simulink model "controller_dev_sg_RCP"  (R2018b)
settings: configuration reference "Active" (kept outside this file)
model workspace (MAT data in the model file):
  m = 1000
undefined symbols (not defined in the file or in its folder): C, tS, TUMHealthStatus, TUMVehicleState
libraries: xpcrtudplib x6, simulink x6, canmsglib x6, etargetslib x5, misc x4, speedgoatlib_IO614 x3, slrtlib x2
(part 2 of 3)

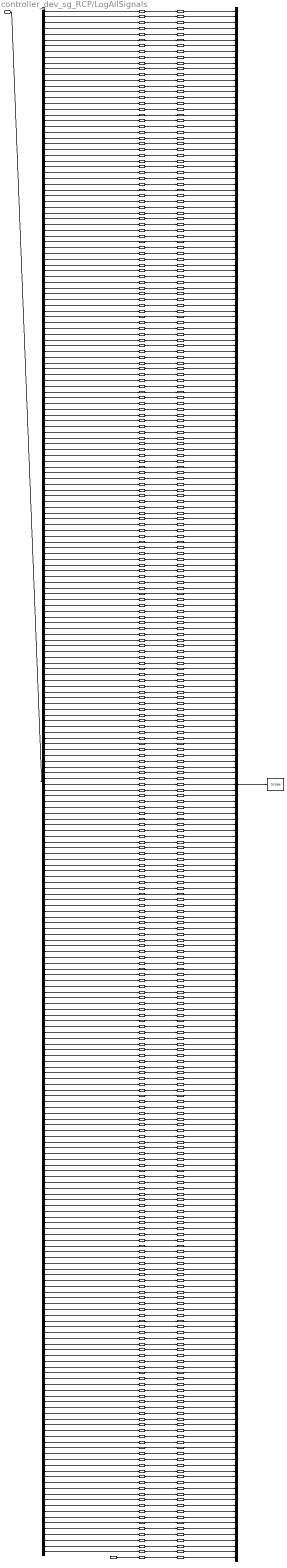
== system controller_dev_sg_RCP/LogAllSignals ==
  debugIn : Inport  OutDataTypeStr=Bus: mvdc_vehicle_dynamics_control_debug
  BusOutput : BusSelector  OutputSignals=ErrorCode,mvdc_path_feedback_debug.BarriersL_x_m,mvdc_path_feedback_debug.BarriersL_y_m,mvdc_path_feedback_debug.BarriersR_x_m,mvdc_path_feedback_debug.BarriersR_y_m,mvdc_path_feedback_debug.LeftDistance_m,mvdc_path_feedback_debug.RightDistance_m,mvdc_path_feedback_debug.Lat_FB_Barriers,mvdc_path_feedback_debug.Lat_FB_Sum_KappaReq_radpm,mvdc_path_feedback_debug.Lat_FB_Position,mvdc_path_feedback_debug.Lat_FB_Heading,mvdc_path_feedback_debug.Lat_LatPosError_m,mvdc_path_feedback_debug.Lat_LatPosError_DerAna_mps,mvdc_path_feedback_debug.Lat_LatPosError_DerNum_mps,mvdc_path_feedback_debug.Lat_FF_Kappa_KappaReq_radpm,mvdc_path_feedback_debug.Lat_FF_FIR_radpm,mvdc_path_feedback_debug.Lat_all_KappaReq_radpm,mvdc_path_matching_debug.PerformanceTrajOK_b,mvdc_path_matching_debug.EmergencyTrajOK_b,mvdc_path_matching_debug.PathPos.s_m,mvdc_path_matching_debug.PathPos.d_m,mvdc_path_matching_debug.PathPos.psi_rad,mvdc_path_matching_debug.ActualPathPoint.LapCnt,mvdc_path_matching_debug.ActualPathPoint.TrajCnt,mvdc_path_matching_debug.ActualPathPoint.s_m,mvdc_path_matching_debug.ActualPathPoint.x_m,mvdc_path_matching_debug.ActualPathPoint.y_m,mvdc_path_matching_debug.ActualPathPoint.psi_rad,mvdc_path_matching_debug.ActualPathPoint.kappa_radpm,mvdc_path_matching_debug.ActualPathPoint.kappaFF_radpm,mvdc_path_matching_debug.ActualPathPoint.v_mps,mvdc_path_matching_debug.ActualPathPoint.ax_mps2,mvdc_path_matching_debug.ActualPathPoint.axFF_mps2,mvdc_path_matching_debug.ActualPathPoint.Delta_rad,mvdc_path_matching_debug.ActualPathPoint.DriveForce_N,mvdc_trajectory_driver_debug.ParkBrakeActive,mvdc_trajectory_driver_debug.DriverStatus,mvdc_trajectory_driver_debug.EnablePathMatching,mvdc_trajectory_driver_debug.EnableDriving,mvdc_trajectory_driver_debug.PathMatchingStatus,mvdc_trajectory_driver_debug.Strategy_Status,mvdc_trajectory_driver_debug.Trajectories_CommsStatus,mvdc_trajectory_driver_debug.Strategy_CommsStatus,mvdc_trajectory_driver_perf.LapTime_s,mvdc_trajectory_driver_perf.e_lateral_m,mvdc_trajectory_driver_perf.eRMS_lateral_m,mvdc_trajectory_driver_perf.ePeak_lateral_m,mvdc_trajectory_driver_perf.e_heading_rad,mvdc_trajectory_driver_perf.eRMS_heading_rad,mvdc_trajectory_driver_perf.ePeak_heading_rad,mvdc_trajectory_driver_perf.e_v_mps,mvdc_trajectory_driver_perf.eRMS_v_mps,mvdc_trajectory_driver_perf.ePeak_v_mps,mvdc_trajectory_driver_perf.e_kappa_radpm,mvdc_trajectory_driver_perf.eRMS_kappa_radpm,mvdc_trajectory_driver_perf.ePeak_kappa_radpm,mvdc_curvvel_tracking_debug.Curv_TargetAy_mps2,mvdc_curvvel_tracking_debug.Curv_all_KappaReq_radpm,mvdc_curvvel_tracking_debug.Curv_FB_Dist_DeltaReq_rad,mvdc_curvvel_tracking_debug.Curv_FB_Diff_DeltaReq_rad,mvdc_curvvel_tracking_debug.Curv_FF_Kappa_DeltaReq_rad,mvdc_curvvel_tracking_debug.Curv_USComp_DeltaReq_rad,mvdc_curvvel_tracking_debug.Curv_CurvError_radpm,mvdc_curvvel_tracking_debug.Curv_TargetCurv_radpm,mvdc_curvvel_tracking_debug.Long_FB_Dist_FxReq_N,mvdc_curvvel_tracking_debug.Long_FF_Dist_FxReq_N,mvdc_curvvel_tracking_debug.Long_FB_VelDiff_FxReq_N,mvdc_curvvel_tracking_debug.Long_FF_Traj_FxReq_N,mvdc_curvvel_tracking_debug.Long_VelError_mps,mvdc_curvvel_tracking_debug.Long_TargetSpeed_mps,mvdc_curvvel_tracking_debug.Long_axTarget_mps2,mvdc_curvvel_tracking_debug.Req_Delta_rad,mvdc_curvvel_tracking_debug.Req_Fx_N,mvdc_curvvel_tracking_debug.ControlState,mvdc_curvvel_tracking_debug.EnableDriving,mvdc_curvvel_tracking_debug.EnableEmergency,mvdc_curvvel_tracking_debug.TCCorrectiveForce_N,mvdc_curvvel_tracking_debug.TCSlipDifference_perc,mvdc_curvvel_tracking_debug.TCProportionalForce_N,mvdc_curvvel_tracking_debug.TCIntegralForce_N,mvdc_curvvel_tracking_debug.MaximumLongForce_N,mvdc_exactlin_feedback_debug.VelocityError_mps,mvdc_exactlin_feedback_debug.LongAccTarget_mps2,mvdc_exactlin_feedback_debug.LatError_m,mvdc_exactlin_feedback_debug.LatErrorDer_mps,mvdc_exactlin_feedback_debug.LatAccTarget_mps2,mvdc_exactlin_feedback_debug.EstimateAlphaF_rad,mvdc_exactlin_feedback_debug.EstimateAlphaR_rad,mvdc_exactlin_feedback_debug.EstimateFyF_N,mvdc_exactlin_feedback_debug.EstimateFyR_N,mvdc_exactlin_feedback_debug.RequestDelta_rad,mvdc_exactlin_feedback_debug.RequestFx_N,mvdc_state_estimation_debug.StateEstimate.SE_Status,mvdc_state_estimation_debug.StateEstimate.SE_State,mvdc_state_estimation_debug.StateEstimate.Pos.x_m,mvdc_state_estimation_debug.StateEstimate.Pos.y_m,mvdc_state_estimation_debug.StateEstimate.Pos.psi_rad,mvdc_state_estimation_debug.StateEstimate.z_m,mvdc_state_estimation_debug.StateEstimate.PosAccuracy,mvdc_state_estimation_debug.StateEstimate.VelAccuracy,mvdc_state_estimation_debug.StateEstimate.dPsi_radps,mvdc_state_estimation_debug.StateEstimate.vx_mps,mvdc_state_estimation_debug.StateEstimate.vy_mps,mvdc_state_estimation_debug.StateEstimate.v_mps,mvdc_state_estimation_debug.StateEstimate.beta_rad,mvdc_state_estimation_debug.StateEstimate.ax_mps2,mvdc_state_estimation_debug.StateEstimate.ay_mps2,mvdc_state_estimation_debug.StateEstimate.psi_vel_rad,mvdc_state_estimation_debug.StateEstimate.kappa_radpm,mvdc_state_estimation_debug.StateEstimate.dBeta_radps,mvdc_state_estimation_debug.StateEstimate.ddPsi_radps2,mvdc_state_estimation_debug.StateEstimate.ax_vel_mps2,mvdc_state_estimation_debug.StateEstimate.ay_vel_mps2,mvdc_state_estimation_debug.StateEstimate.lambdaFL_perc,mvdc_state_estimation_debug.StateEstimate.lambdaFR_perc,mvdc_state_estimation_debug.StateEstimate.lambdaRL_perc,mvdc_state_estimation_debug.StateEstimate.lambdaRR_perc,mvdc_state_estimation_debug.StateEstimate.alphaFL_rad,mvdc_state_estimation_debug.StateEstimate.alphaFR_rad,mvdc_state_estimation_debug.StateEstimate.alphaRL_rad,mvdc_state_estimation_debug.StateEstimate.alphaRR_rad,mvdc_state_estimation_debug.StateEstimate.DiffFRAlpha_rad,mvdc_state_estimation_debug.Residuals.res_xLoc1_m,mvdc_state_estimation_debug.Residuals.res_yLoc1_m,mvdc_state_estimation_debug.Residuals.res_psiLoc1_rad,mvdc_state_estimation_debug.Residuals.res_xLoc2_m,mvdc_state_estimation_debug.Residuals.res_yLoc2_m,mvdc_state_estimation_debug.Residuals.res_psiLoc2_rad,mvdc_state_estimation_debug.Residuals.res_vxVel1_mps,mvdc_state_estimation_debug.Residuals.res_vyVel1_mps,mvdc_state_estimation_debug.Residuals.res_vxVel2_mps,mvdc_state_estimation_debug.Residuals.res_vyVel2_mps,mvdc_state_estimation_debug.Residuals.res_dPsi1_radps,mvdc_state_estimation_debug.Residuals.res_dPsi2_radps,mvdc_state_estimation_debug.Residuals.res_sLoc1_m,mvdc_state_estimation_debug.Residuals.res_dLoc1_m,mvdc_state_estimation_debug.Residuals.res_sLoc2_m,mvdc_state_estimation_debug.Residuals.res_dLoc2_m,mvdc_state_estimation_debug.Diagnosis.valid_Loc1_b,mvdc_state_estimation_debug.Diagnosis.valid_Loc2_b,mvdc_state_estimation_debug.Diagnosis.valid_Vel1_b,mvdc_state_estimation_debug.Diagnosis.valid_Vel2_b,mvdc_state_estimation_debug.Diagnosis.valid_IMU1_b,mvdc_state_estimation_debug.Diagnosis.valid_IMU2_b,mvdc_state_estimation_debug.Diagnosis.fail_Loc1_b,mvdc_state_estimation_debug.Diagnosis.fail_Loc2_b,mvdc_state_estimation_debug.Diagnosis.fail_Vel1_b,mvdc_state_estimation_debug.Diagnosis.fail_Vel2_b,mvdc_state_estimation_debug.Diagnosis.fail_IMU1_b,mvdc_state_estimation_debug.Diagnosis.fail_IMU2_b,mvdc_state_estimation_debug.Odom.Position.x_m,mvdc_state_estimation_debug.Odom.Position.y_m,mvdc_state_estimation_debug.Odom.Position.psi_rad,mvdc_state_estimation_debug.Odom.Valid_b,mloc_statemachine_debug.Hardware_Status,mloc_statemachine_debug.AIDriver_Status,mloc_statemachine_debug.ParkBrakeApplied_b,mloc_statemachine_debug.VehicleReady2Drive,mloc_statemachine_debug.StateEstimation_Status,mloc_statemachine_debug.VehicleSafeStandstill,mloc_statemachine_debug.Driver_Status,mloc_statemachine_debug.VehicleUnresponsive,mloc_statemachine_debug.TUMVehicleState,mloc_statemachine_debug.EnableSensorFusion,mloc_statemachine_debug.EnableControlOutputs,mloc_statemachine_debug.EnableDriver,mloc_statemachine_debug.EnableHardEmergencyBrake,mloc_statemachine_debug.RequestControl,mloc_diag_vehicle_debug.VehicleUnstable_b,mloc_diag_vehicle_debug.EstimatedCurrentPower_W,mloc_diag_vehicle_debug.EstimatedRequestedPower_W,mvdc_mue_estimation_rt_debug.Position.x_m,mvdc_mue_estimation_rt_debug.Position.y_m,mvdc_mue_estimation_rt_debug.Position.psi_rad,mvdc_mue_estimation_rt_debug.mue_estimation_AxleF,mvdc_mue_estimation_rt_debug.mue_estimation_AxleR,mvdc_mue_estimation_delay_debug.Position.x_m,mvdc_mue_estimation_delay_debug.Position.y_m,mvdc_mue_estimation_delay_debug.Position.psi_rad,mvdc_mue_estimation_delay_debug.FX_VehDynFL_N,mvdc_mue_estimation_delay_debug.FX_VehDynFR_N,mvdc_mue_estimation_delay_debug.FX_VehDynRL_N,mvdc_mue_estimation_delay_debug.FX_VehDynRR_N,mvdc_mue_estimation_delay_debug.FY_VehDynFL_N,mvdc_mue_estimation_delay_debug.FY_VehDynFR_N,mvdc_mue_estimation_delay_debug.FY_VehDynRL_N,mvdc_mue_estimation_delay_debug.FY_VehDynRR_N,mvdc_mue_estimation_delay_debug.FZ_VehDynFL_N,mvdc_mue_estimation_delay_debug.FZ_VehDynFR_N,mvdc_mue_estimation_delay_debug.FZ_VehDynRL_N,mvdc_mue_estimation_delay_debug.FZ_VehDynRR_N,mvdc_mue_estimation_delay_debug.FX_MFtireforceFL_N,mvdc_mue_estimation_delay_debug.FY_MFtireforceFL_N,mvdc_mue_estimation_delay_debug.FX_MFtireforceFLmax_N,mvdc_mue_estimation_delay_debug.FY_MFtireforceFLmax_N,mvdc_mue_estimation_delay_debug.FX_MFtireforceFR_N,mvdc_mue_estimation_delay_debug.FY_MFtireforceFR_N,mvdc_mue_estimation_delay_debug.FX_MFtireforceFRmax_N,mvdc_mue_estimation_delay_debug.FY_MFtireforceFRmax_N,mvdc_mue_estimation_delay_debug.FX_MFtireforceRL_N,mvdc_mue_estimation_delay_debug.FY_MFtireforceRL_N,mvdc_mue_estimation_delay_debug.FX_MFtireforceRLmax_N,mvdc_mue_estimation_delay_debug.FY_MFtireforceRLmax_N,mvdc_mue_estimation_delay_debug.FX_MFtireforceRR_N,mvdc_mue_estimation_delay_debug.FY_MFtireforceRR_N,mvdc_mue_estimation_delay_debug.FX_MFtireforceRRmax_N,mvdc_mue_estimation_delay_debug.FY_MFtireforceRRmax_N,mvdc_mue_estimation_delay_debug.TRFP_est_FLx,mvdc_mue_estimation_delay_debug.TRFP_est_FLy,mvdc_mue_estimation_delay_debug.TRFP_est_FRx,mvdc_mue_estimation_delay_debug.TRFP_est_FRy,mvdc_mue_estimation_delay_debug.TRFP_est_RLx,mvdc_mue_estimation_delay_debug.TRFP_est_RLy,mvdc_mue_estimation_delay_debug.TRFP_est_RRx,mvdc_mue_estimation_delay_debug.TRFP_est_RRy,VehicleSensorData.Tz_Powertrain_Nm,VehicleSensorData.Fx_Powertrain_N,VehicleSensorData.T_WheelFL_Nm,VehicleSensorData.T_WheelFR_Nm,VehicleSensorData.T_WheelRL_Nm,VehicleSensorData.T_WheelRR_Nm,VehicleSensorData.Delta_Wheel_rad,VehicleSensorData.p_BrakeF_bar,VehicleSensorData.p_BrakeR_bar,VehicleSensorData.omega_WheelFL_radps,VehicleSensorData.omega_WheelFR_radps,VehicleSensorData.omega_WheelRL_radps,VehicleSensorData.omega_WheelRR_radps,VehicleSensorData.valid_Wheelspeeds_b,VehicleSensorData.x_Loc1_m,VehicleSensorData.y_Loc1_m,VehicleSensorData.z_Loc1_m,VehicleSensorData.phi_RollAngleLoc1_rad,VehicleSensorData.theta_PitchAngleLoc1_rad,VehicleSensorData.psi_YawAngleLoc1_rad,VehicleSensorData.t_EstimateLoc1_s,VehicleSensorData.valid_Loc1_b,VehicleSensorData.accuracy_Loc1,VehicleSensorData.x_Loc2_m,VehicleSensorData.y_Loc2_m,VehicleSensorData.z_Loc2_m,VehicleSensorData.phi_RollAngleLoc2_rad,VehicleSensorData.theta_PitchAngleLoc2_rad,VehicleSensorData.psi_YawAngleLoc2_rad,VehicleSensorData.t_EstimateLoc2_s,VehicleSensorData.valid_Loc2_b,VehicleSensorData.accuracy_Loc2,VehicleSensorData.vx_CoGVel1_mps,VehicleSensorData.vy_CoGVel1_mps,VehicleSensorData.valid_Vel1_b,VehicleSensorData.vx_CoGVel2_mps,VehicleSensorData.vy_CoGVel2_mps,VehicleSensorData.valid_Vel2_b,VehicleSensorData.ax_CoGIMU1_mps2,VehicleSensorData.ay_CoGIMU1_mps2,VehicleSensorData.az_CoGIMU1_mps2,VehicleSensorData.dPhi_RollRateIMU1_radps,VehicleSensorData.dTheta_PitchRateIMU1_radps,VehicleSensorData.dPsi_YawRateIMU1_radps,VehicleSensorData.valid_IMU1_b,VehicleSensorData.ax_CoGIMU2_mps2,VehicleSensorData.ay_CoGIMU2_mps2,VehicleSensorData.az_CoGIMU2_mps2,VehicleSensorData.dPhi_RollRateIMU2_radps,VehicleSensorData.dTheta_PitchRateIMU2_radps,VehicleSensorData.dPsi_YawRateIMU2_radps,VehicleSensorData.valid_IMU2_b,Time_s
  Convert{1..269} (269 alike) : DataTypeConversion  OutDataTypeStr=single  SaturateOnIntegerOverflow=on  RndMeth=Zero
  LoggingScope : slrtlib/Displays and Logging/Scope   scopeno=1  scopetype=File  autostart=on  viewmode=Graphical redraw  formatstr='%15.6f'  grid=on  ylimits=[0,0]  nosamples=32  noprepostsamples=0  interleave=1  triggermode=FreeRun  triggersignal=1  trigsignalfromport=off  triggerlevel=0.0  triggerslope=Either  triggerscope=1  triggersample=0  filename=sgdebug<%>.dat  mode=Commit  writesize=512  autorestart=on  dynamicfilemode=on  maxwritefilesize=512*2048^2
  Mux : Mux  Inputs=269
  TET : slrtlib/Target Management/Execution Parameters/Task Execution Time   ts=0.004
      settings: SourceProductName=Simulink Real-Time  SourceProductBaseCode=XP
  debug_ErrorCode : SignalConversion  OverrideOpt=off
  debug_TET_s : SignalConversion  OverrideOpt=off
  debug_Time_s : SignalConversion  OverrideOpt=off
  debug_VehicleSensorData_Delta_Wheel_rad : SignalConversion  OverrideOpt=off
  debug_VehicleSensorData_Fx_Powertrain_N : SignalConversion  OverrideOpt=off
  debug_VehicleSensorData_T_WheelFL_Nm : SignalConversion  OverrideOpt=off
  debug_VehicleSensorData_T_WheelFR_Nm : SignalConversion  OverrideOpt=off
  debug_VehicleSensorData_T_WheelRL_Nm : SignalConversion  OverrideOpt=off
  debug_VehicleSensorData_T_WheelRR_Nm : SignalConversion  OverrideOpt=off
  debug_VehicleSensorData_Tz_Powertrain_Nm : SignalConversion  OverrideOpt=off
  debug_VehicleSensorData_accuracy_Loc1 : SignalConversion  OverrideOpt=off
  debug_VehicleSensorData_accuracy_Loc2 : SignalConversion  OverrideOpt=off
  debug_VehicleSensorData_ax_CoGIMU1_mps2 : SignalConversion  OverrideOpt=off
  debug_VehicleSensorData_ax_CoGIMU2_mps2 : SignalConversion  OverrideOpt=off
  debug_VehicleSensorData_ay_CoGIMU1_mps2 : SignalConversion  OverrideOpt=off
  debug_VehicleSensorData_ay_CoGIMU2_mps2 : SignalConversion  OverrideOpt=off
  debug_VehicleSensorData_az_CoGIMU1_mps2 : SignalConversion  OverrideOpt=off
  debug_VehicleSensorData_az_CoGIMU2_mps2 : SignalConversion  OverrideOpt=off
  debug_VehicleSensorData_dPhi_RollRateIMU1_radps : SignalConversion  OverrideOpt=off
  debug_VehicleSensorData_dPhi_RollRateIMU2_radps : SignalConversion  OverrideOpt=off
  debug_VehicleSensorData_dPsi_YawRateIMU1_radps : SignalConversion  OverrideOpt=off
  debug_VehicleSensorData_dPsi_YawRateIMU2_radps : SignalConversion  OverrideOpt=off
  debug_VehicleSensorData_dTheta_PitchRateIMU1_radps : SignalConversion  OverrideOpt=off
  debug_VehicleSensorData_dTheta_PitchRateIMU2_radps : SignalConversion  OverrideOpt=off
  debug_VehicleSensorData_omega_WheelFL_radps : SignalConversion  OverrideOpt=off
  debug_VehicleSensorData_omega_WheelFR_radps : SignalConversion  OverrideOpt=off
  debug_VehicleSensorData_omega_WheelRL_radps : SignalConversion  OverrideOpt=off
  debug_VehicleSensorData_omega_WheelRR_radps : SignalConversion  OverrideOpt=off
  debug_VehicleSensorData_p_BrakeF_bar : SignalConversion  OverrideOpt=off
  debug_VehicleSensorData_p_BrakeR_bar : SignalConversion  OverrideOpt=off
  debug_VehicleSensorData_phi_RollAngleLoc1_rad : SignalConversion  OverrideOpt=off
  debug_VehicleSensorData_phi_RollAngleLoc2_rad : SignalConversion  OverrideOpt=off
  debug_VehicleSensorData_psi_YawAngleLoc1_rad : SignalConversion  OverrideOpt=off
  debug_VehicleSensorData_psi_YawAngleLoc2_rad : SignalConversion  OverrideOpt=off
  debug_VehicleSensorData_t_EstimateLoc1_s : SignalConversion  OverrideOpt=off
  debug_VehicleSensorData_t_EstimateLoc2_s : SignalConversion  OverrideOpt=off
  debug_VehicleSensorData_theta_PitchAngleLoc1_rad : SignalConversion  OverrideOpt=off
  debug_VehicleSensorData_theta_PitchAngleLoc2_rad : SignalConversion  OverrideOpt=off
  debug_VehicleSensorData_valid_IMU1_b : SignalConversion  OverrideOpt=off
  debug_VehicleSensorData_valid_IMU2_b : SignalConversion  OverrideOpt=off
  debug_VehicleSensorData_valid_Loc1_b : SignalConversion  OverrideOpt=off
  debug_VehicleSensorData_valid_Loc2_b : SignalConversion  OverrideOpt=off
  debug_VehicleSensorData_valid_Vel1_b : SignalConversion  OverrideOpt=off
  debug_VehicleSensorData_valid_Vel2_b : SignalConversion  OverrideOpt=off
  debug_VehicleSensorData_valid_Wheelspeeds_b : SignalConversion  OverrideOpt=off
  debug_VehicleSensorData_vx_CoGVel1_mps : SignalConversion  OverrideOpt=off
  debug_VehicleSensorData_vx_CoGVel2_mps : SignalConversion  OverrideOpt=off
  debug_VehicleSensorData_vy_CoGVel1_mps : SignalConversion  OverrideOpt=off
  debug_VehicleSensorData_vy_CoGVel2_mps : SignalConversion  OverrideOpt=off
  debug_VehicleSensorData_x_Loc1_m : SignalConversion  OverrideOpt=off
  debug_VehicleSensorData_x_Loc2_m : SignalConversion  OverrideOpt=off
  debug_VehicleSensorData_y_Loc1_m : SignalConversion  OverrideOpt=off
  debug_VehicleSensorData_y_Loc2_m : SignalConversion  OverrideOpt=off
  debug_VehicleSensorData_z_Loc1_m : SignalConversion  OverrideOpt=off
  debug_VehicleSensorData_z_Loc2_m : SignalConversion  OverrideOpt=off
  debug_mloc_diag_vehicle_debug_EstimatedCurrentPower_W : SignalConversion  OverrideOpt=off
  debug_mloc_diag_vehicle_debug_EstimatedRequestedPower_W : SignalConversion  OverrideOpt=off
  debug_mloc_diag_vehicle_debug_VehicleUnstable_b : SignalConversion  OverrideOpt=off
  debug_mloc_statemachine_debug_AIDriver_Status : SignalConversion  OverrideOpt=off
  debug_mloc_statemachine_debug_Driver_Status : SignalConversion  OverrideOpt=off
  debug_mloc_statemachine_debug_EnableControlOutputs : SignalConversion  OverrideOpt=off
  debug_mloc_statemachine_debug_EnableDriver : SignalConversion  OverrideOpt=off
  debug_mloc_statemachine_debug_EnableHardEmergencyBrake : SignalConversion  OverrideOpt=off
  debug_mloc_statemachine_debug_EnableSensorFusion : SignalConversion  OverrideOpt=off
  debug_mloc_statemachine_debug_Hardware_Status : SignalConversion  OverrideOpt=off
  debug_mloc_statemachine_debug_ParkBrakeApplied_b : SignalConversion  OverrideOpt=off
  debug_mloc_statemachine_debug_RequestControl : SignalConversion  OverrideOpt=off
  debug_mloc_statemachine_debug_StateEstimation_Status : SignalConversion  OverrideOpt=off
  debug_mloc_statemachine_debug_TUMVehicleState : SignalConversion  OverrideOpt=off
  debug_mloc_statemachine_debug_VehicleReady2Drive : SignalConversion  OverrideOpt=off
  debug_mloc_statemachine_debug_VehicleSafeStandstill : SignalConversion  OverrideOpt=off
  debug_mloc_statemachine_debug_VehicleUnresponsive : SignalConversion  OverrideOpt=off
  debug_mvdc_curvvel_tracking_debug_ControlState : SignalConversion  OverrideOpt=off
  debug_mvdc_curvvel_tracking_debug_Curv_CurvError_radpm : SignalConversion  OverrideOpt=off
  debug_mvdc_curvvel_tracking_debug_Curv_FB_Diff_DeltaReq_rad : SignalConversion  OverrideOpt=off
  debug_mvdc_curvvel_tracking_debug_Curv_FB_Dist_DeltaReq_rad : SignalConversion  OverrideOpt=off
  debug_mvdc_curvvel_tracking_debug_Curv_FF_Kappa_DeltaReq_rad : SignalConversion  OverrideOpt=off
  debug_mvdc_curvvel_tracking_debug_Curv_TargetAy_mps2 : SignalConversion  OverrideOpt=off
  debug_mvdc_curvvel_tracking_debug_Curv_TargetCurv_radpm : SignalConversion  OverrideOpt=off
  debug_mvdc_curvvel_tracking_debug_Curv_USComp_DeltaReq_rad : SignalConversion  OverrideOpt=off
  debug_mvdc_curvvel_tracking_debug_Curv_all_KappaReq_radpm : SignalConversion  OverrideOpt=off
  debug_mvdc_curvvel_tracking_debug_EnableDriving : SignalConversion  OverrideOpt=off
  debug_mvdc_curvvel_tracking_debug_EnableEmergency : SignalConversion  OverrideOpt=off
  debug_mvdc_curvvel_tracking_debug_Long_FB_Dist_FxReq_N : SignalConversion  OverrideOpt=off
  debug_mvdc_curvvel_tracking_debug_Long_FB_VelDiff_FxReq_N : SignalConversion  OverrideOpt=off
  debug_mvdc_curvvel_tracking_debug_Long_FF_Dist_FxReq_N : SignalConversion  OverrideOpt=off
  debug_mvdc_curvvel_tracking_debug_Long_FF_Traj_FxReq_N : SignalConversion  OverrideOpt=off
  debug_mvdc_curvvel_tracking_debug_Long_TargetSpeed_mps : SignalConversion  OverrideOpt=off
  debug_mvdc_curvvel_tracking_debug_Long_VelError_mps : SignalConversion  OverrideOpt=off
  debug_mvdc_curvvel_tracking_debug_Long_axTarget_mps2 : SignalConversion  OverrideOpt=off
  debug_mvdc_curvvel_tracking_debug_MaximumLongForce_N : SignalConversion  OverrideOpt=off
  debug_mvdc_curvvel_tracking_debug_Req_Delta_rad : SignalConversion  OverrideOpt=off
  debug_mvdc_curvvel_tracking_debug_Req_Fx_N : SignalConversion  OverrideOpt=off
  debug_mvdc_curvvel_tracking_debug_TCCorrectiveForce_N : SignalConversion  OverrideOpt=off
  debug_mvdc_curvvel_tracking_debug_TCIntegralForce_N : SignalConversion  OverrideOpt=off
  debug_mvdc_curvvel_tracking_debug_TCProportionalForce_N : SignalConversion  OverrideOpt=off
  debug_mvdc_curvvel_tracking_debug_TCSlipDifference_perc : SignalConversion  OverrideOpt=off
  debug_mvdc_exactlin_feedback_debug_EstimateAlphaF_rad : SignalConversion  OverrideOpt=off
  debug_mvdc_exactlin_feedback_debug_EstimateAlphaR_rad : SignalConversion  OverrideOpt=off
  debug_mvdc_exactlin_feedback_debug_EstimateFyF_N : SignalConversion  OverrideOpt=off
  debug_mvdc_exactlin_feedback_debug_EstimateFyR_N : SignalConversion  OverrideOpt=off
  debug_mvdc_exactlin_feedback_debug_LatAccTarget_mps2 : SignalConversion  OverrideOpt=off
  debug_mvdc_exactlin_feedback_debug_LatErrorDer_mps : SignalConversion  OverrideOpt=off
  debug_mvdc_exactlin_feedback_debug_LatError_m : SignalConversion  OverrideOpt=off
  debug_mvdc_exactlin_feedback_debug_LongAccTarget_mps2 : SignalConversion  OverrideOpt=off
  debug_mvdc_exactlin_feedback_debug_RequestDelta_rad : SignalConversion  OverrideOpt=off
  debug_mvdc_exactlin_feedback_debug_RequestFx_N : SignalConversion  OverrideOpt=off
  debug_mvdc_exactlin_feedback_debug_VelocityError_mps : SignalConversion  OverrideOpt=off
  debug_mvdc_mue_estimation_delay_debug_FX_MFtireforceFL_N : SignalConversion  OverrideOpt=off
  debug_mvdc_mue_estimation_delay_debug_FX_MFtireforceFLmax_N : SignalConversion  OverrideOpt=off
  debug_mvdc_mue_estimation_delay_debug_FX_MFtireforceFR_N : SignalConversion  OverrideOpt=off
  debug_mvdc_mue_estimation_delay_debug_FX_MFtireforceFRmax_N : SignalConversion  OverrideOpt=off
  debug_mvdc_mue_estimation_delay_debug_FX_MFtireforceRL_N : SignalConversion  OverrideOpt=off
  debug_mvdc_mue_estimation_delay_debug_FX_MFtireforceRLmax_N : SignalConversion  OverrideOpt=off
  debug_mvdc_mue_estimation_delay_debug_FX_MFtireforceRR_N : SignalConversion  OverrideOpt=off
  debug_mvdc_mue_estimation_delay_debug_FX_MFtireforceRRmax_N : SignalConversion  OverrideOpt=off
  debug_mvdc_mue_estimation_delay_debug_FX_VehDynFL_N : SignalConversion  OverrideOpt=off
  debug_mvdc_mue_estimation_delay_debug_FX_VehDynFR_N : SignalConversion  OverrideOpt=off
  debug_mvdc_mue_estimation_delay_debug_FX_VehDynRL_N : SignalConversion  OverrideOpt=off
  debug_mvdc_mue_estimation_delay_debug_FX_VehDynRR_N : SignalConversion  OverrideOpt=off
  debug_mvdc_mue_estimation_delay_debug_FY_MFtireforceFL_N : SignalConversion  OverrideOpt=off
  debug_mvdc_mue_estimation_delay_debug_FY_MFtireforceFLmax_N : SignalConversion  OverrideOpt=off
  debug_mvdc_mue_estimation_delay_debug_FY_MFtireforceFR_N : SignalConversion  OverrideOpt=off
  debug_mvdc_mue_estimation_delay_debug_FY_MFtireforceFRmax_N : SignalConversion  OverrideOpt=off
  debug_mvdc_mue_estimation_delay_debug_FY_MFtireforceRL_N : SignalConversion  OverrideOpt=off
  debug_mvdc_mue_estimation_delay_debug_FY_MFtireforceRLmax_N : SignalConversion  OverrideOpt=off
  debug_mvdc_mue_estimation_delay_debug_FY_MFtireforceRR_N : SignalConversion  OverrideOpt=off
  debug_mvdc_mue_estimation_delay_debug_FY_MFtireforceRRmax_N : SignalConversion  OverrideOpt=off
  debug_mvdc_mue_estimation_delay_debug_FY_VehDynFL_N : SignalConversion  OverrideOpt=off
  debug_mvdc_mue_estimation_delay_debug_FY_VehDynFR_N : SignalConversion  OverrideOpt=off
  debug_mvdc_mue_estimation_delay_debug_FY_VehDynRL_N : SignalConversion  OverrideOpt=off
  debug_mvdc_mue_estimation_delay_debug_FY_VehDynRR_N : SignalConversion  OverrideOpt=off
  debug_mvdc_mue_estimation_delay_debug_FZ_VehDynFL_N : SignalConversion  OverrideOpt=off
  debug_mvdc_mue_estimation_delay_debug_FZ_VehDynFR_N : SignalConversion  OverrideOpt=off
  debug_mvdc_mue_estimation_delay_debug_FZ_VehDynRL_N : SignalConversion  OverrideOpt=off
  debug_mvdc_mue_estimation_delay_debug_FZ_VehDynRR_N : SignalConversion  OverrideOpt=off
  debug_mvdc_mue_estimation_delay_debug_Position_psi_rad : SignalConversion  OverrideOpt=off
  debug_mvdc_mue_estimation_delay_debug_Position_x_m : SignalConversion  OverrideOpt=off
  debug_mvdc_mue_estimation_delay_debug_Position_y_m : SignalConversion  OverrideOpt=off
  debug_mvdc_mue_estimation_delay_debug_TRFP_est_FLx : SignalConversion  OverrideOpt=off
  debug_mvdc_mue_estimation_delay_debug_TRFP_est_FLy : SignalConversion  OverrideOpt=off
  debug_mvdc_mue_estimation_delay_debug_TRFP_est_FRx : SignalConversion  OverrideOpt=off
  debug_mvdc_mue_estimation_delay_debug_TRFP_est_FRy : SignalConversion  OverrideOpt=off
  debug_mvdc_mue_estimation_delay_debug_TRFP_est_RLx : SignalConversion  OverrideOpt=off
  debug_mvdc_mue_estimation_delay_debug_TRFP_est_RLy : SignalConversion  OverrideOpt=off
  debug_mvdc_mue_estimation_delay_debug_TRFP_est_RRx : SignalConversion  OverrideOpt=off
  debug_mvdc_mue_estimation_delay_debug_TRFP_est_RRy : SignalConversion  OverrideOpt=off
  debug_mvdc_mue_estimation_rt_debug_Position_psi_rad : SignalConversion  OverrideOpt=off
  debug_mvdc_mue_estimation_rt_debug_Position_x_m : SignalConversion  OverrideOpt=off
  debug_mvdc_mue_estimation_rt_debug_Position_y_m : SignalConversion  OverrideOpt=off
  debug_mvdc_mue_estimation_rt_debug_mue_estimation_AxleF : SignalConversion  OverrideOpt=off
  debug_mvdc_mue_estimation_rt_debug_mue_estimation_AxleR : SignalConversion  OverrideOpt=off
  debug_mvdc_path_feedback_debug_BarriersL_x_m : SignalConversion  OverrideOpt=off
  debug_mvdc_path_feedback_debug_BarriersL_y_m : SignalConversion  OverrideOpt=off
  debug_mvdc_path_feedback_debug_BarriersR_x_m : SignalConversion  OverrideOpt=off
  debug_mvdc_path_feedback_debug_BarriersR_y_m : SignalConversion  OverrideOpt=off
  debug_mvdc_path_feedback_debug_Lat_FB_Barriers : SignalConversion  OverrideOpt=off
  debug_mvdc_path_feedback_debug_Lat_FB_Heading : SignalConversion  OverrideOpt=off
  debug_mvdc_path_feedback_debug_Lat_FB_Position : SignalConversion  OverrideOpt=off
  debug_mvdc_path_feedback_debug_Lat_FB_Sum_KappaReq_radpm : SignalConversion  OverrideOpt=off
  debug_mvdc_path_feedback_debug_Lat_FF_FIR_radpm : SignalConversion  OverrideOpt=off
  debug_mvdc_path_feedback_debug_Lat_FF_Kappa_KappaReq_radpm : SignalConversion  OverrideOpt=off
  debug_mvdc_path_feedback_debug_Lat_LatPosError_DerAna_mps : SignalConversion  OverrideOpt=off
  debug_mvdc_path_feedback_debug_Lat_LatPosError_DerNum_mps : SignalConversion  OverrideOpt=off
  debug_mvdc_path_feedback_debug_Lat_LatPosError_m : SignalConversion  OverrideOpt=off
  debug_mvdc_path_feedback_debug_Lat_all_KappaReq_radpm : SignalConversion  OverrideOpt=off
  debug_mvdc_path_feedback_debug_LeftDistance_m : SignalConversion  OverrideOpt=off
  debug_mvdc_path_feedback_debug_RightDistance_m : SignalConversion  OverrideOpt=off
  debug_mvdc_path_matching_debug_ActualPathPoint_Delta_rad : SignalConversion  OverrideOpt=off
  debug_mvdc_path_matching_debug_ActualPathPoint_DriveForce_N : SignalConversion  OverrideOpt=off
  debug_mvdc_path_matching_debug_ActualPathPoint_LapCnt : SignalConversion  OverrideOpt=off
  debug_mvdc_path_matching_debug_ActualPathPoint_TrajCnt : SignalConversion  OverrideOpt=off
  debug_mvdc_path_matching_debug_ActualPathPoint_axFF_mps2 : SignalConversion  OverrideOpt=off
  debug_mvdc_path_matching_debug_ActualPathPoint_ax_mps2 : SignalConversion  OverrideOpt=off
  debug_mvdc_path_matching_debug_ActualPathPoint_kappaFF_radpm : SignalConversion  OverrideOpt=off
  debug_mvdc_path_matching_debug_ActualPathPoint_kappa_radpm : SignalConversion  OverrideOpt=off
  debug_mvdc_path_matching_debug_ActualPathPoint_psi_rad : SignalConversion  OverrideOpt=off
  debug_mvdc_path_matching_debug_ActualPathPoint_s_m : SignalConversion  OverrideOpt=off
  debug_mvdc_path_matching_debug_ActualPathPoint_v_mps : SignalConversion  OverrideOpt=off
  debug_mvdc_path_matching_debug_ActualPathPoint_x_m : SignalConversion  OverrideOpt=off
  debug_mvdc_path_matching_debug_ActualPathPoint_y_m : SignalConversion  OverrideOpt=off
  debug_mvdc_path_matching_debug_EmergencyTrajOK_b : SignalConversion  OverrideOpt=off
  debug_mvdc_path_matching_debug_PathPos_d_m : SignalConversion  OverrideOpt=off
  debug_mvdc_path_matching_debug_PathPos_psi_rad : SignalConversion  OverrideOpt=off
  debug_mvdc_path_matching_debug_PathPos_s_m : SignalConversion  OverrideOpt=off
  debug_mvdc_path_matching_debug_PerformanceTrajOK_b : SignalConversion  OverrideOpt=off
  debug_mvdc_state_estimation_debug_Diagnosis_fail_IMU1_b : SignalConversion  OverrideOpt=off
  debug_mvdc_state_estimation_debug_Diagnosis_fail_IMU2_b : SignalConversion  OverrideOpt=off
  debug_mvdc_state_estimation_debug_Diagnosis_fail_Loc1_b : SignalConversion  OverrideOpt=off
  debug_mvdc_state_estimation_debug_Diagnosis_fail_Loc2_b : SignalConversion  OverrideOpt=off
  debug_mvdc_state_estimation_debug_Diagnosis_fail_Vel1_b : SignalConversion  OverrideOpt=off
  debug_mvdc_state_estimation_debug_Diagnosis_fail_Vel2_b : SignalConversion  OverrideOpt=off
  debug_mvdc_state_estimation_debug_Diagnosis_valid_IMU1_b : SignalConversion  OverrideOpt=off
  debug_mvdc_state_estimation_debug_Diagnosis_valid_IMU2_b : SignalConversion  OverrideOpt=off
  debug_mvdc_state_estimation_debug_Diagnosis_valid_Loc1_b : SignalConversion  OverrideOpt=off
  debug_mvdc_state_estimation_debug_Diagnosis_valid_Loc2_b : SignalConversion  OverrideOpt=off
  debug_mvdc_state_estimation_debug_Diagnosis_valid_Vel1_b : SignalConversion  OverrideOpt=off
  debug_mvdc_state_estimation_debug_Diagnosis_valid_Vel2_b : SignalConversion  OverrideOpt=off
  debug_mvdc_state_estimation_debug_Odom_Position_psi_rad : SignalConversion  OverrideOpt=off
  debug_mvdc_state_estimation_debug_Odom_Position_x_m : SignalConversion  OverrideOpt=off
  debug_mvdc_state_estimation_debug_Odom_Position_y_m : SignalConversion  OverrideOpt=off
  debug_mvdc_state_estimation_debug_Odom_Valid_b : SignalConversion  OverrideOpt=off
  debug_mvdc_state_estimation_debug_Residuals_res_dLoc1_m : SignalConversion  OverrideOpt=off
  debug_mvdc_state_estimation_debug_Residuals_res_dLoc2_m : SignalConversion  OverrideOpt=off
  debug_mvdc_state_estimation_debug_Residuals_res_dPsi1_radps : SignalConversion  OverrideOpt=off
  debug_mvdc_state_estimation_debug_Residuals_res_dPsi2_radps : SignalConversion  OverrideOpt=off
  debug_mvdc_state_estimation_debug_Residuals_res_psiLoc1_rad : SignalConversion  OverrideOpt=off
  debug_mvdc_state_estimation_debug_Residuals_res_psiLoc2_rad : SignalConversion  OverrideOpt=off
  debug_mvdc_state_estimation_debug_Residuals_res_sLoc1_m : SignalConversion  OverrideOpt=off
  debug_mvdc_state_estimation_debug_Residuals_res_sLoc2_m : SignalConversion  OverrideOpt=off
  debug_mvdc_state_estimation_debug_Residuals_res_vxVel1_mps : SignalConversion  OverrideOpt=off
  debug_mvdc_state_estimation_debug_Residuals_res_vxVel2_mps : SignalConversion  OverrideOpt=off
  debug_mvdc_state_estimation_debug_Residuals_res_vyVel1_mps : SignalConversion  OverrideOpt=off
  debug_mvdc_state_estimation_debug_Residuals_res_vyVel2_mps : SignalConversion  OverrideOpt=off
  debug_mvdc_state_estimation_debug_Residuals_res_xLoc1_m : SignalConversion  OverrideOpt=off
  debug_mvdc_state_estimation_debug_Residuals_res_xLoc2_m : SignalConversion  OverrideOpt=off
  debug_mvdc_state_estimation_debug_Residuals_res_yLoc1_m : SignalConversion  OverrideOpt=off
  debug_mvdc_state_estimation_debug_Residuals_res_yLoc2_m : SignalConversion  OverrideOpt=off
  debug_mvdc_state_estimation_debug_StateEstimate_DiffFRAlpha_rad : SignalConversion  OverrideOpt=off
  debug_mvdc_state_estimation_debug_StateEstimate_PosAccuracy : SignalConversion  OverrideOpt=off
  debug_mvdc_state_estimation_debug_StateEstimate_Pos_psi_rad : SignalConversion  OverrideOpt=off
  debug_mvdc_state_estimation_debug_StateEstimate_Pos_x_m : SignalConversion  OverrideOpt=off
  debug_mvdc_state_estimation_debug_StateEstimate_Pos_y_m : SignalConversion  OverrideOpt=off
  debug_mvdc_state_estimation_debug_StateEstimate_SE_State : SignalConversion  OverrideOpt=off
  debug_mvdc_state_estimation_debug_StateEstimate_SE_Status : SignalConversion  OverrideOpt=off
  debug_mvdc_state_estimation_debug_StateEstimate_VelAccuracy : SignalConversion  OverrideOpt=off
  debug_mvdc_state_estimation_debug_StateEstimate_alphaFL_rad : SignalConversion  OverrideOpt=off
  debug_mvdc_state_estimation_debug_StateEstimate_alphaFR_rad : SignalConversion  OverrideOpt=off
  debug_mvdc_state_estimation_debug_StateEstimate_alphaRL_rad : SignalConversion  OverrideOpt=off
  debug_mvdc_state_estimation_debug_StateEstimate_alphaRR_rad : SignalConversion  OverrideOpt=off
  debug_mvdc_state_estimation_debug_StateEstimate_ax_mps2 : SignalConversion  OverrideOpt=off
  debug_mvdc_state_estimation_debug_StateEstimate_ax_vel_mps2 : SignalConversion  OverrideOpt=off
  debug_mvdc_state_estimation_debug_StateEstimate_ay_mps2 : SignalConversion  OverrideOpt=off
  debug_mvdc_state_estimation_debug_StateEstimate_ay_vel_mps2 : SignalConversion  OverrideOpt=off
  debug_mvdc_state_estimation_debug_StateEstimate_beta_rad : SignalConversion  OverrideOpt=off
  debug_mvdc_state_estimation_debug_StateEstimate_dBeta_radps : SignalConversion  OverrideOpt=off
  debug_mvdc_state_estimation_debug_StateEstimate_dPsi_radps : SignalConversion  OverrideOpt=off
  debug_mvdc_state_estimation_debug_StateEstimate_ddPsi_radps2 : SignalConversion  OverrideOpt=off
  debug_mvdc_state_estimation_debug_StateEstimate_kappa_radpm : SignalConversion  OverrideOpt=off
  debug_mvdc_state_estimation_debug_StateEstimate_lambdaFL_perc : SignalConversion  OverrideOpt=off
  debug_mvdc_state_estimation_debug_StateEstimate_lambdaFR_perc : SignalConversion  OverrideOpt=off
  debug_mvdc_state_estimation_debug_StateEstimate_lambdaRL_perc : SignalConversion  OverrideOpt=off
  debug_mvdc_state_estimation_debug_StateEstimate_lambdaRR_perc : SignalConversion  OverrideOpt=off
  debug_mvdc_state_estimation_debug_StateEstimate_psi_vel_rad : SignalConversion  OverrideOpt=off
  debug_mvdc_state_estimation_debug_StateEstimate_v_mps : SignalConversion  OverrideOpt=off
  debug_mvdc_state_estimation_debug_StateEstimate_vx_mps : SignalConversion  OverrideOpt=off
  debug_mvdc_state_estimation_debug_StateEstimate_vy_mps : SignalConversion  OverrideOpt=off
  debug_mvdc_state_estimation_debug_StateEstimate_z_m : SignalConversion  OverrideOpt=off
  debug_mvdc_trajectory_driver_debug_DriverStatus : SignalConversion  OverrideOpt=off
  debug_mvdc_trajectory_driver_debug_EnableDriving : SignalConversion  OverrideOpt=off
  debug_mvdc_trajectory_driver_debug_EnablePathMatching : SignalConversion  OverrideOpt=off
  debug_mvdc_trajectory_driver_debug_ParkBrakeActive : SignalConversion  OverrideOpt=off
  debug_mvdc_trajectory_driver_debug_PathMatchingStatus : SignalConversion  OverrideOpt=off
  debug_mvdc_trajectory_driver_debug_Strategy_CommsStatus : SignalConversion  OverrideOpt=off
  debug_mvdc_trajectory_driver_debug_Strategy_Status : SignalConversion  OverrideOpt=off
  debug_mvdc_trajectory_driver_debug_Trajectories_CommsStatus : SignalConversion  OverrideOpt=off
  debug_mvdc_trajectory_driver_perf_LapTime_s : SignalConversion  OverrideOpt=off
  debug_mvdc_trajectory_driver_perf_ePeak_heading_rad : SignalConversion  OverrideOpt=off
  debug_mvdc_trajectory_driver_perf_ePeak_kappa_radpm : SignalConversion  OverrideOpt=off
  debug_mvdc_trajectory_driver_perf_ePeak_lateral_m : SignalConversion  OverrideOpt=off
  debug_mvdc_trajectory_driver_perf_ePeak_v_mps : SignalConversion  OverrideOpt=off
  debug_mvdc_trajectory_driver_perf_eRMS_heading_rad : SignalConversion  OverrideOpt=off
  debug_mvdc_trajectory_driver_perf_eRMS_kappa_radpm : SignalConversion  OverrideOpt=off
  debug_mvdc_trajectory_driver_perf_eRMS_lateral_m : SignalConversion  OverrideOpt=off
  debug_mvdc_trajectory_driver_perf_eRMS_v_mps : SignalConversion  OverrideOpt=off
  debug_mvdc_trajectory_driver_perf_e_heading_rad : SignalConversion  OverrideOpt=off
  debug_mvdc_trajectory_driver_perf_e_kappa_radpm : SignalConversion  OverrideOpt=off
  debug_mvdc_trajectory_driver_perf_e_lateral_m : SignalConversion  OverrideOpt=off
  debug_mvdc_trajectory_driver_perf_e_v_mps : SignalConversion  OverrideOpt=off
  wires:
  BusOutput/76 -> Convert76/1  "<EnableEmergency>"
  Convert247/1 -> debug_VehicleSensorData_accuracy_Loc2/1
  BusOutput/247 -> Convert247/1  "<accuracy_Loc2>"
  debug_mvdc_mue_estimation_delay_debug_FZ_VehDynRR_N/1 -> Mux/191
  debug_mvdc_mue_estimation_rt_debug_mue_estimation_AxleR/1 -> Mux/176
  BusOutput/146 -> Convert146/1  "<fail_Loc2_b>"
  debug_mvdc_exactlin_feedback_debug_RequestFx_N/1 -> Mux/92
  BusOutput/245 -> Convert245/1  "<t_EstimateLoc2_s>"
  Convert37/1 -> debug_mvdc_trajectory_driver_debug_DriverStatus/1
  BusOutput/163 -> Convert163/1  "<TUMVehicleState>"
  Convert153/1 -> debug_mvdc_state_estimation_debug_Odom_Position_psi_rad/1
  BusOutput/201 -> Convert201/1  "<FY_MFtireforceRL_N>"
  debug_VehicleSensorData_y_Loc2_m/1 -> Mux/240
  debug_mvdc_state_estimation_debug_StateEstimate_ax_vel_mps2/1 -> Mux/112
  Convert201/1 -> debug_mvdc_mue_estimation_delay_debug_FY_MFtireforceRL_N/1
  Convert188/1 -> debug_mvdc_mue_estimation_delay_debug_FZ_VehDynFL_N/1
  BusOutput/155 -> Convert155/1  "<Hardware_Status>"
  debug_VehicleSensorData_valid_Loc1_b/1 -> Mux/237
  BusOutput/100 -> Convert100/1  "<VelAccuracy>"
  debug_mvdc_mue_estimation_delay_debug_FX_MFtireforceRL_N/1 -> Mux/200
  Convert198/1 -> debug_mvdc_mue_estimation_delay_debug_FX_MFtireforceFRmax_N/1
  Convert104/1 -> debug_mvdc_state_estimation_debug_StateEstimate_v_mps/1
  Convert168/1 -> debug_mloc_statemachine_debug_RequestControl/1
  debug_mvdc_mue_estimation_delay_debug_TRFP_est_RLy/1 -> Mux/213
  BusOutput/143 -> Convert143/1  "<valid_IMU1_b>"
  Convert110/1 -> debug_mvdc_state_estimation_debug_StateEstimate_dBeta_radps/1
  debug_mvdc_mue_estimation_delay_debug_FX_MFtireforceRLmax_N/1 -> Mux/202
  Convert162/1 -> debug_mloc_statemachine_debug_VehicleUnresponsive/1
  BusOutput/235 -> Convert235/1  "<psi_YawAngleLoc1_rad>"
  BusOutput/156 -> Convert156/1  "<AIDriver_Status>"
  debug_mvdc_curvvel_tracking_debug_Curv_FF_Kappa_DeltaReq_rad/1 -> Mux/61
  Convert74/1 -> debug_mvdc_curvvel_tracking_debug_ControlState/1
  BusOutput/239 -> Convert239/1  "<x_Loc2_m>"
  Convert235/1 -> debug_VehicleSensorData_psi_YawAngleLoc1_rad/1
  debug_mvdc_mue_estimation_delay_debug_FY_MFtireforceFR_N/1 -> Mux/197
  Convert157/1 -> debug_mloc_statemachine_debug_ParkBrakeApplied_b/1
  BusOutput/228 -> Convert228/1  "<omega_WheelRR_radps>"
  Convert148/1 -> debug_mvdc_state_estimation_debug_Diagnosis_fail_Vel2_b/1
  Convert6/1 -> debug_mvdc_path_feedback_debug_LeftDistance_m/1
  BusOutput/50 -> Convert50/1  "<ePeak_heading_rad>"
  debug_VehicleSensorData_valid_Loc2_b/1 -> Mux/246
  BusOutput/104 -> Convert104/1  "<v_mps>"
  debug_VehicleSensorData_x_Loc1_m/1 -> Mux/230
  debug_VehicleSensorData_omega_WheelFR_radps/1 -> Mux/226
  Convert246/1 -> debug_VehicleSensorData_valid_Loc2_b/1
  BusOutput/227 -> Convert227/1  "<omega_WheelRL_radps>"
  debug_mvdc_path_matching_debug_ActualPathPoint_ax_mps2/1 -> Mux/32
  Convert154/1 -> debug_mvdc_state_estimation_debug_Odom_Valid_b/1
  BusOutput/232 -> Convert232/1  "<z_Loc1_m>"
  BusOutput/186 -> Convert186/1  "<FY_VehDynRL_N>"
  Convert225/1 -> debug_VehicleSensorData_omega_WheelFL_radps/1
  Convert35/1 -> debug_mvdc_path_matching_debug_ActualPathPoint_DriveForce_N/1
  debug_VehicleSensorData_omega_WheelFL_radps/1 -> Mux/225
  debug_mvdc_state_estimation_debug_Diagnosis_fail_Loc2_b/1 -> Mux/146
  BusOutput/148 -> Convert148/1  "<fail_Vel2_b>"
  debug_mvdc_curvvel_tracking_debug_Curv_all_KappaReq_radpm/1 -> Mux/58
  BusOutput/224 -> Convert224/1  "<p_BrakeR_bar>"
  BusOutput/233 -> Convert233/1  "<phi_RollAngleLoc1_rad>"
  debug_mvdc_mue_estimation_delay_debug_FY_MFtireforceRRmax_N/1 -> Mux/207
  Convert170/1 -> debug_mloc_diag_vehicle_debug_EstimatedCurrentPower_W/1
  Convert223/1 -> debug_VehicleSensorData_p_BrakeF_bar/1
  Convert133/1 -> debug_mvdc_state_estimation_debug_Residuals_res_dPsi1_radps/1
  BusOutput/211 -> Convert211/1  "<TRFP_est_FRy>"
  debug_VehicleSensorData_omega_WheelRR_radps/1 -> Mux/228
  BusOutput/193 -> Convert193/1  "<FY_MFtireforceFL_N>"
  BusOutput/221 -> Convert221/1  "<T_WheelRR_Nm>"
  Convert222/1 -> debug_VehicleSensorData_Delta_Wheel_rad/1
  Convert180/1 -> debug_mvdc_mue_estimation_delay_debug_FX_VehDynFL_N/1
  debug_mvdc_state_estimation_debug_StateEstimate_VelAccuracy/1 -> Mux/100
  BusOutput/199 -> Convert199/1  "<FY_MFtireforceFRmax_N>"
  Convert96/1 -> debug_mvdc_state_estimation_debug_StateEstimate_Pos_y_m/1
  debug_mloc_statemachine_debug_VehicleSafeStandstill/1 -> Mux/160
  debug_VehicleSensorData_T_WheelFL_Nm/1 -> Mux/218
  BusOutput/218 -> Convert218/1  "<T_WheelFL_Nm>"
  BusOutput/217 -> Convert217/1  "<Fx_Powertrain_N>"
  BusOutput/51 -> Convert51/1  "<e_v_mps>"
  Convert214/1 -> debug_mvdc_mue_estimation_delay_debug_TRFP_est_RRx/1
  debug_mvdc_state_estimation_debug_Residuals_res_vxVel2_mps/1 -> Mux/131
  BusOutput/153 -> Convert153/1  "<psi_rad>"
  debug_mvdc_mue_estimation_delay_debug_Position_y_m/1 -> Mux/178
  Convert213/1 -> debug_mvdc_mue_estimation_delay_debug_TRFP_est_RLy/1
  BusOutput/214 -> Convert214/1  "<TRFP_est_RRx>"
  BusOutput/125 -> Convert125/1  "<res_psiLoc1_rad>"
  Convert217/1 -> debug_VehicleSensorData_Fx_Powertrain_N/1
  BusOutput/215 -> Convert215/1  "<TRFP_est_RRy>"
  BusOutput/205 -> Convert205/1  "<FY_MFtireforceRR_N>"
  debug_mvdc_mue_estimation_delay_debug_TRFP_est_FRy/1 -> Mux/211
  Convert211/1 -> debug_mvdc_mue_estimation_delay_debug_TRFP_est_FRy/1
  BusOutput/210 -> Convert210/1  "<TRFP_est_FRx>"
  Convert191/1 -> debug_mvdc_mue_estimation_delay_debug_FZ_VehDynRR_N/1
  BusOutput/207 -> Convert207/1  "<FY_MFtireforceRRmax_N>"
  BusOutput/98 -> Convert98/1  "<z_m>"
  debug_mvdc_mue_estimation_rt_debug_Position_psi_rad/1 -> Mux/174
  debug_mvdc_mue_estimation_delay_debug_TRFP_est_FLx/1 -> Mux/208
  debug_mvdc_state_estimation_debug_StateEstimate_lambdaFR_perc/1 -> Mux/115
  Convert186/1 -> debug_mvdc_mue_estimation_delay_debug_FY_VehDynRL_N/1
  BusOutput/206 -> Convert206/1  "<FX_MFtireforceRRmax_N>"
  Convert166/1 -> debug_mloc_statemachine_debug_EnableDriver/1
  BusOutput/189 -> Convert189/1  "<FZ_VehDynFR_N>"
  debug_mvdc_mue_estimation_delay_debug_FZ_VehDynFL_N/1 -> Mux/188
  debug_mvdc_mue_estimation_delay_debug_FX_MFtireforceRRmax_N/1 -> Mux/206
  debug_mvdc_mue_estimation_delay_debug_FY_MFtireforceRR_N/1 -> Mux/205
  BusOutput/249 -> Convert249/1  "<vy_CoGVel1_mps>"
  Convert199/1 -> debug_mvdc_mue_estimation_delay_debug_FY_MFtireforceFRmax_N/1
  BusOutput/132 -> Convert132/1  "<res_vyVel2_mps>"
  BusOutput/222 -> Convert222/1  "<Delta_Wheel_rad>"
  Convert224/1 -> debug_VehicleSensorData_p_BrakeR_bar/1
  debug_VehicleSensorData_vx_CoGVel1_mps/1 -> Mux/248
  Convert161/1 -> debug_mloc_statemachine_debug_Driver_Status/1
  BusOutput/145 -> Convert145/1  "<fail_Loc1_b>"
  debug_VehicleSensorData_z_Loc2_m/1 -> Mux/241
  Convert245/1 -> debug_VehicleSensorData_t_EstimateLoc2_s/1
  BusOutput/248 -> Convert248/1  "<vx_CoGVel1_mps>"
  debug_mvdc_path_feedback_debug_BarriersL_x_m/1 -> Mux/2
  Convert128/1 -> debug_mvdc_state_estimation_debug_Residuals_res_psiLoc2_rad/1
  Convert231/1 -> debug_VehicleSensorData_y_Loc1_m/1
  debug_VehicleSensorData_accuracy_Loc2/1 -> Mux/247
  BusOutput/234 -> Convert234/1  "<theta_PitchAngleLoc1_rad>"
  BusOutput/208 -> Convert208/1  "<TRFP_est_FLx>"
  Convert15/1 -> debug_mvdc_path_feedback_debug_Lat_FF_Kappa_KappaReq_radpm/1
  BusOutput/213 -> Convert213/1  "<TRFP_est_RLy>"
  BusOutput/229 -> Convert229/1  "<valid_Wheelspeeds_b>"
  Convert178/1 -> debug_mvdc_mue_estimation_delay_debug_Position_y_m/1
  BusOutput/181 -> Convert181/1  "<FX_VehDynFR_N>"
  BusOutput/266 -> Convert266/1  "<dPsi_YawRateIMU2_radps>"
  BusOutput/19 -> Convert19/1  "<EmergencyTrajOK_b>"
  BusOutput/144 -> Convert144/1  "<valid_IMU2_b>"
  BusOutput/238 -> Convert238/1  "<accuracy_Loc1>"
  debug_mvdc_state_estimation_debug_Residuals_res_vyVel2_mps/1 -> Mux/132
  BusOutput/246 -> Convert246/1  "<valid_Loc2_b>"
  BusOutput/243 -> Convert243/1  "<theta_PitchAngleLoc2_rad>"
  BusOutput/255 -> Convert255/1  "<ay_CoGIMU1_mps2>"
  BusOutput/195 -> Convert195/1  "<FY_MFtireforceFLmax_N>"
  debug_VehicleSensorData_T_WheelFR_Nm/1 -> Mux/219
  Convert218/1 -> debug_VehicleSensorData_T_WheelFL_Nm/1
  Convert147/1 -> debug_mvdc_state_estimation_debug_Diagnosis_fail_Vel1_b/1
  Convert253/1 -> debug_VehicleSensorData_valid_Vel2_b/1
  debug_VehicleSensorData_Delta_Wheel_rad/1 -> Mux/222
  BusOutput/128 -> Convert128/1  "<res_psiLoc2_rad>"
  Convert36/1 -> debug_mvdc_trajectory_driver_debug_ParkBrakeActive/1
  BusOutput/216 -> Convert216/1  "<Tz_Powertrain_Nm>"
  debug_mvdc_state_estimation_debug_StateEstimate_ay_mps2/1 -> Mux/107
  debug_VehicleSensorData_Fx_Powertrain_N/1 -> Mux/217
  BusOutput/225 -> Convert225/1  "<omega_WheelFL_radps>"
  Convert266/1 -> debug_VehicleSensorData_dPsi_YawRateIMU2_radps/1
  Convert267/1 -> debug_VehicleSensorData_valid_IMU2_b/1
  debug_VehicleSensorData_dPhi_RollRateIMU2_radps/1 -> Mux/264
  Convert242/1 -> debug_VehicleSensorData_phi_RollAngleLoc2_rad/1
  BusOutput/97 -> Convert97/1  "<psi_rad>"
  Convert256/1 -> debug_VehicleSensorData_az_CoGIMU1_mps2/1
  debug_mvdc_trajectory_driver_perf_eRMS_v_mps/1 -> Mux/52
  BusOutput/264 -> Convert264/1  "<dPhi_RollRateIMU2_radps>"
  Convert192/1 -> debug_mvdc_mue_estimation_delay_debug_FX_MFtireforceFL_N/1
  debug_VehicleSensorData_ax_CoGIMU1_mps2/1 -> Mux/254
  Convert123/1 -> debug_mvdc_state_estimation_debug_Residuals_res_xLoc1_m/1
  Convert240/1 -> debug_VehicleSensorData_y_Loc2_m/1
  BusOutput/262 -> Convert262/1  "<ay_CoGIMU2_mps2>"
  debug_mvdc_state_estimation_debug_StateEstimate_DiffFRAlpha_rad/1 -> Mux/122
  BusOutput/165 -> Convert165/1  "<EnableControlOutputs>"
  Convert200/1 -> debug_mvdc_mue_estimation_delay_debug_FX_MFtireforceRL_N/1
  BusOutput/3 -> Convert3/1  "<BarriersL_y_m>"
  debug_VehicleSensorData_t_EstimateLoc2_s/1 -> Mux/245
  BusOutput/263 -> Convert263/1  "<az_CoGIMU2_mps2>"
  debug_VehicleSensorData_theta_PitchAngleLoc2_rad/1 -> Mux/243
  Convert261/1 -> debug_VehicleSensorData_ax_CoGIMU2_mps2/1
  Convert258/1 -> debug_VehicleSensorData_dTheta_PitchRateIMU1_radps/1
  debug_mloc_statemachine_debug_VehicleUnresponsive/1 -> Mux/162
  Convert238/1 -> debug_VehicleSensorData_accuracy_Loc1/1
  debug_VehicleSensorData_valid_IMU1_b/1 -> Mux/260
  debug_mloc_statemachine_debug_AIDriver_Status/1 -> Mux/156
  BusOutput/80 -> Convert80/1  "<TCIntegralForce_N>"
  Convert230/1 -> debug_VehicleSensorData_x_Loc1_m/1
  BusOutput/252 -> Convert252/1  "<vy_CoGVel2_mps>"
  debug_VehicleSensorData_t_EstimateLoc1_s/1 -> Mux/236
  Convert134/1 -> debug_mvdc_state_estimation_debug_Residuals_res_dPsi2_radps/1
  BusOutput/198 -> Convert198/1  "<FX_MFtireforceFRmax_N>"
  Convert255/1 -> debug_VehicleSensorData_ay_CoGIMU1_mps2/1
  Convert52/1 -> debug_mvdc_trajectory_driver_perf_eRMS_v_mps/1
  BusOutput/191 -> Convert191/1  "<FZ_VehDynRR_N>"
  BusOutput/259 -> Convert259/1  "<dPsi_YawRateIMU1_radps>"
  Convert227/1 -> debug_VehicleSensorData_omega_WheelRL_radps/1
  debug_mvdc_curvvel_tracking_debug_TCIntegralForce_N/1 -> Mux/80
  BusOutput/160 -> Convert160/1  "<VehicleSafeStandstill>"
  BusOutput/257 -> Convert257/1  "<dPhi_RollRateIMU1_radps>"
  BusOutput/151 -> Convert151/1  "<x_m>"
  BusOutput/192 -> Convert192/1  "<FX_MFtireforceFL_N>"
  debug_mvdc_mue_estimation_delay_debug_FX_VehDynFL_N/1 -> Mux/180
  Convert42/1 -> debug_mvdc_trajectory_driver_debug_Trajectories_CommsStatus/1
  debug_VehicleSensorData_vy_CoGVel2_mps/1 -> Mux/252
  Convert239/1 -> debug_VehicleSensorData_x_Loc2_m/1
  BusOutput/7 -> Convert7/1  "<RightDistance_m>"
  Convert251/1 -> debug_VehicleSensorData_vx_CoGVel2_mps/1
  BusOutput/251 -> Convert251/1  "<vx_CoGVel2_mps>"
  Convert252/1 -> debug_VehicleSensorData_vy_CoGVel2_mps/1
  debug_VehicleSensorData_valid_Vel2_b/1 -> Mux/253
  Convert229/1 -> debug_VehicleSensorData_valid_Wheelspeeds_b/1
  debug_mloc_diag_vehicle_debug_EstimatedRequestedPower_W/1 -> Mux/171
  debug_mvdc_path_feedback_debug_Lat_FF_Kappa_KappaReq_radpm/1 -> Mux/15
  debug_mvdc_trajectory_driver_debug_Trajectories_CommsStatus/1 -> Mux/42
  debug_mvdc_mue_estimation_delay_debug_TRFP_est_RLx/1 -> Mux/212
  Convert228/1 -> debug_VehicleSensorData_omega_WheelRR_radps/1
  debug_mloc_statemachine_debug_ParkBrakeApplied_b/1 -> Mux/157
  debug_VehicleSensorData_vy_CoGVel1_mps/1 -> Mux/249
  debug_mvdc_mue_estimation_delay_debug_FY_MFtireforceFLmax_N/1 -> Mux/195
  Convert233/1 -> debug_VehicleSensorData_phi_RollAngleLoc1_rad/1
  Convert206/1 -> debug_mvdc_mue_estimation_delay_debug_FX_MFtireforceRRmax_N/1
  Convert250/1 -> debug_VehicleSensorData_valid_Vel1_b/1
  Convert263/1 -> debug_VehicleSensorData_az_CoGIMU2_mps2/1
  debug_VehicleSensorData_az_CoGIMU1_mps2/1 -> Mux/256
  Convert158/1 -> debug_mloc_statemachine_debug_VehicleReady2Drive/1
  Convert264/1 -> debug_VehicleSensorData_dPhi_RollRateIMU2_radps/1
  BusOutput/174 -> Convert174/1  "<psi_rad>"
  Convert244/1 -> debug_VehicleSensorData_psi_YawAngleLoc2_rad/1
  BusOutput/203 -> Convert203/1  "<FY_MFtireforceRLmax_N>"
  Convert243/1 -> debug_VehicleSensorData_theta_PitchAngleLoc2_rad/1
  debug_mloc_statemachine_debug_EnableDriver/1 -> Mux/166
  debug_VehicleSensorData_y_Loc1_m/1 -> Mux/231
  debug_VehicleSensorData_az_CoGIMU2_mps2/1 -> Mux/263
  BusOutput/194 -> Convert194/1  "<FX_MFtireforceFLmax_N>"
  Convert49/1 -> debug_mvdc_trajectory_driver_perf_eRMS_heading_rad/1
  Mux/1 -> LoggingScope/1
  Convert260/1 -> debug_VehicleSensorData_valid_IMU1_b/1
  debug_mvdc_mue_estimation_delay_debug_FY_MFtireforceRLmax_N/1 -> Mux/203
  BusOutput/240 -> Convert240/1  "<y_Loc2_m>"
  BusOutput/117 -> Convert117/1  "<lambdaRR_perc>"
  Convert80/1 -> debug_mvdc_curvvel_tracking_debug_TCIntegralForce_N/1
  TET/1 -> Convert269/1
  Convert45/1 -> debug_mvdc_trajectory_driver_perf_e_lateral_m/1
  Convert234/1 -> debug_VehicleSensorData_theta_PitchAngleLoc1_rad/1
  BusOutput/92 -> Convert92/1  "<RequestFx_N>"
  Convert189/1 -> debug_mvdc_mue_estimation_delay_debug_FZ_VehDynFR_N/1
  Convert61/1 -> debug_mvdc_curvvel_tracking_debug_Curv_FF_Kappa_DeltaReq_rad/1
  debug_mvdc_state_estimation_debug_StateEstimate_alphaRL_rad/1 -> Mux/120
  debug_mvdc_mue_estimation_delay_debug_FY_VehDynRL_N/1 -> Mux/186
  BusOutput/46 -> Convert46/1  "<eRMS_lateral_m>"
  BusOutput/230 -> Convert230/1  "<x_Loc1_m>"
  Convert44/1 -> debug_mvdc_trajectory_driver_perf_LapTime_s/1
  debug_VehicleSensorData_ax_CoGIMU2_mps2/1 -> Mux/261
  debug_VehicleSensorData_dTheta_PitchRateIMU2_radps/1 -> Mux/265
  BusOutput/133 -> Convert133/1  "<res_dPsi1_radps>"
  Convert57/1 -> debug_mvdc_curvvel_tracking_debug_Curv_TargetAy_mps2/1
  BusOutput/183 -> Convert183/1  "<FX_VehDynRR_N>"
  debug_VehicleSensorData_p_BrakeR_bar/1 -> Mux/224
  Convert46/1 -> debug_mvdc_trajectory_driver_perf_eRMS_lateral_m/1
  Convert187/1 -> debug_mvdc_mue_estimation_delay_debug_FY_VehDynRR_N/1
  BusOutput/184 -> Convert184/1  "<FY_VehDynFL_N>"
  Convert77/1 -> debug_mvdc_curvvel_tracking_debug_TCCorrectiveForce_N/1
  BusOutput/182 -> Convert182/1  "<FX_VehDynRL_N>"
  debug_mvdc_trajectory_driver_perf_ePeak_kappa_radpm/1 -> Mux/56
  debug_mvdc_mue_estimation_delay_debug_FY_VehDynFL_N/1 -> Mux/184
  debug_mvdc_mue_estimation_delay_debug_Position_x_m/1 -> Mux/177
  BusOutput/81 -> Convert81/1  "<MaximumLongForce_N>"
  BusOutput/185 -> Convert185/1  "<FY_VehDynFR_N>"
  debug_mvdc_mue_estimation_delay_debug_FX_MFtireforceRR_N/1 -> Mux/204
  Convert73/1 -> debug_mvdc_curvvel_tracking_debug_Req_Fx_N/1
  debug_VehicleSensorData_phi_RollAngleLoc1_rad/1 -> Mux/233
  Convert173/1 -> debug_mvdc_mue_estimation_rt_debug_Position_y_m/1
  debug_mvdc_mue_estimation_rt_debug_Position_y_m/1 -> Mux/173
  debug_mvdc_trajectory_driver_debug_EnableDriving/1 -> Mux/39
  Convert194/1 -> debug_mvdc_mue_estimation_delay_debug_FX_MFtireforceFLmax_N/1
  BusOutput/109 -> Convert109/1  "<kappa_radpm>"
  BusOutput/254 -> Convert254/1  "<ax_CoGIMU1_mps2>"
  BusOutput/111 -> Convert111/1  "<ddPsi_radps2>"
  BusOutput/170 -> Convert170/1  "<EstimatedCurrentPower_W>"
  Convert16/1 -> debug_mvdc_path_feedback_debug_Lat_FF_FIR_radpm/1
  debug_mvdc_curvvel_tracking_debug_Curv_TargetCurv_radpm/1 -> Mux/64
  debug_mloc_diag_vehicle_debug_VehicleUnstable_b/1 -> Mux/169
  debug_Time_s/1 -> Mux/268
  debug_mloc_statemachine_debug_EnableHardEmergencyBrake/1 -> Mux/167
  BusOutput/118 -> Convert118/1  "<alphaFL_rad>"
  Convert226/1 -> debug_VehicleSensorData_omega_WheelFR_radps/1
  Convert216/1 -> debug_VehicleSensorData_Tz_Powertrain_Nm/1
  BusOutput/179 -> Convert179/1  "<psi_rad>"
  BusOutput/168 -> Convert168/1  "<RequestControl>"
  debug_mvdc_mue_estimation_delay_debug_FX_VehDynRL_N/1 -> Mux/182
  debug_mloc_statemachine_debug_RequestControl/1 -> Mux/168
  debug_mvdc_state_estimation_debug_StateEstimate_vy_mps/1 -> Mux/103
  Convert164/1 -> debug_mloc_statemachine_debug_EnableSensorFusion/1
  Convert167/1 -> debug_mloc_statemachine_debug_EnableHardEmergencyBrake/1
  BusOutput/147 -> Convert147/1  "<fail_Vel1_b>"
  debug_mloc_statemachine_debug_EnableControlOutputs/1 -> Mux/165
  debug_mvdc_state_estimation_debug_Residuals_res_dLoc1_m/1 -> Mux/136
  debug_mloc_statemachine_debug_EnableSensorFusion/1 -> Mux/164
  BusOutput/164 -> Convert164/1  "<EnableSensorFusion>"
  Convert177/1 -> debug_mvdc_mue_estimation_delay_debug_Position_x_m/1
  Convert58/1 -> debug_mvdc_curvvel_tracking_debug_Curv_all_KappaReq_radpm/1
  Convert156/1 -> debug_mloc_statemachine_debug_AIDriver_Status/1
  BusOutput/139 -> Convert139/1  "<valid_Loc1_b>"
  BusOutput/171 -> Convert171/1  "<EstimatedRequestedPower_W>"
  Convert160/1 -> debug_mloc_statemachine_debug_VehicleSafeStandstill/1
  Convert109/1 -> debug_mvdc_state_estimation_debug_StateEstimate_kappa_radpm/1
  Convert159/1 -> debug_mloc_statemachine_debug_StateEstimation_Status/1
  BusOutput/154 -> Convert154/1  "<Valid_b>"
  BusOutput/142 -> Convert142/1  "<valid_Vel2_b>"
  Convert155/1 -> debug_mloc_statemachine_debug_Hardware_Status/1
  debug_mvdc_state_estimation_debug_Odom_Valid_b/1 -> Mux/154
  debug_mvdc_path_matching_debug_PathPos_d_m/1 -> Mux/21
  debug_mvdc_mue_estimation_delay_debug_FX_VehDynFR_N/1 -> Mux/181
  BusOutput/172 -> Convert172/1  "<x_m>"
  Convert202/1 -> debug_mvdc_mue_estimation_delay_debug_FX_MFtireforceRLmax_N/1
  BusOutput/127 -> Convert127/1  "<res_yLoc2_m>"
  Convert190/1 -> debug_mvdc_mue_estimation_delay_debug_FZ_VehDynRL_N/1
  Convert184/1 -> debug_mvdc_mue_estimation_delay_debug_FY_VehDynFL_N/1
  debug_mvdc_trajectory_driver_debug_Strategy_CommsStatus/1 -> Mux/43
  BusOutput/197 -> Convert197/1  "<FY_MFtireforceFR_N>"
  BusOutput/219 -> Convert219/1  "<T_WheelFR_Nm>"
  BusOutput/178 -> Convert178/1  "<y_m>"
  Convert70/1 -> debug_mvdc_curvvel_tracking_debug_Long_TargetSpeed_mps/1
  BusOutput/200 -> Convert200/1  "<FX_MFtireforceRL_N>"
  BusOutput/86 -> Convert86/1  "<LatAccTarget_mps2>"
  Convert40/1 -> debug_mvdc_trajectory_driver_debug_PathMatchingStatus/1
  BusOutput/63 -> Convert63/1  "<Curv_CurvError_radpm>"
  Convert221/1 -> debug_VehicleSensorData_T_WheelRR_Nm/1
  BusOutput/180 -> Convert180/1  "<FX_VehDynFL_N>"
  Convert269/1 -> debug_TET_s/1
  Convert196/1 -> debug_mvdc_mue_estimation_delay_debug_FX_MFtireforceFR_N/1
  Convert185/1 -> debug_mvdc_mue_estimation_delay_debug_FY_VehDynFR_N/1
  BusOutput/157 -> Convert157/1  "<ParkBrakeApplied_b>"
  BusOutput/158 -> Convert158/1  "<VehicleReady2Drive>"
  Convert195/1 -> debug_mvdc_mue_estimation_delay_debug_FY_MFtireforceFLmax_N/1
  debug_mloc_statemachine_debug_Hardware_Status/1 -> Mux/155
  Convert265/1 -> debug_VehicleSensorData_dTheta_PitchRateIMU2_radps/1
  Convert176/1 -> debug_mvdc_mue_estimation_rt_debug_mue_estimation_AxleR/1
  Convert60/1 -> debug_mvdc_curvvel_tracking_debug_Curv_FB_Diff_DeltaReq_rad/1
  Convert171/1 -> debug_mloc_diag_vehicle_debug_EstimatedRequestedPower_W/1
  Convert10/1 -> debug_mvdc_path_feedback_debug_Lat_FB_Position/1
  BusOutput/150 -> Convert150/1  "<fail_IMU2_b>"
  debug_mvdc_state_estimation_debug_Diagnosis_valid_Vel1_b/1 -> Mux/141
  debug_mvdc_state_estimation_debug_Diagnosis_fail_Vel1_b/1 -> Mux/147
  debug_mvdc_curvvel_tracking_debug_Curv_FB_Dist_DeltaReq_rad/1 -> Mux/59
  BusOutput/65 -> Convert65/1  "<Long_FB_Dist_FxReq_N>"
  debug_mvdc_path_feedback_debug_Lat_LatPosError_DerNum_mps/1 -> Mux/14
  BusOutput/267 -> Convert267/1  "<valid_IMU2_b>"
  BusOutput/58 -> Convert58/1  "<Curv_all_KappaReq_radpm>"
  Convert62/1 -> debug_mvdc_curvvel_tracking_debug_Curv_USComp_DeltaReq_rad/1
  Convert59/1 -> debug_mvdc_curvvel_tracking_debug_Curv_FB_Dist_DeltaReq_rad/1
  debug_mvdc_trajectory_driver_perf_e_v_mps/1 -> Mux/51
  Convert259/1 -> debug_VehicleSensorData_dPsi_YawRateIMU1_radps/1
  BusOutput/59 -> Convert59/1  "<Curv_FB_Dist_DeltaReq_rad>"
  debug_mvdc_trajectory_driver_perf_e_kappa_radpm/1 -> Mux/54
  BusOutput/28 -> Convert28/1  "<psi_rad>"
  Convert63/1 -> debug_mvdc_curvvel_tracking_debug_Curv_CurvError_radpm/1
  debug_mvdc_trajectory_driver_perf_eRMS_kappa_radpm/1 -> Mux/55
  BusOutput/52 -> Convert52/1  "<eRMS_v_mps>"
  debug_VehicleSensorData_psi_YawAngleLoc2_rad/1 -> Mux/244
  Convert150/1 -> debug_mvdc_state_estimation_debug_Diagnosis_fail_IMU2_b/1
  BusOutput/57 -> Convert57/1  "<Curv_TargetAy_mps2>"
  debug_mvdc_mue_estimation_delay_debug_FY_VehDynFR_N/1 -> Mux/185
  debug_mvdc_trajectory_driver_perf_e_heading_rad/1 -> Mux/48
  Convert47/1 -> debug_mvdc_trajectory_driver_perf_ePeak_lateral_m/1
  debug_VehicleSensorData_Tz_Powertrain_Nm/1 -> Mux/216
  Convert48/1 -> debug_mvdc_trajectory_driver_perf_e_heading_rad/1
  debug_VehicleSensorData_ay_CoGIMU2_mps2/1 -> Mux/262
  Convert132/1 -> debug_mvdc_state_estimation_debug_Residuals_res_vyVel2_mps/1
  Convert39/1 -> debug_mvdc_trajectory_driver_debug_EnableDriving/1
  BusOutput/42 -> Convert42/1  "<Trajectories_CommsStatus>"
  debug_VehicleSensorData_dPsi_YawRateIMU2_radps/1 -> Mux/266
  BusOutput/43 -> Convert43/1  "<Strategy_CommsStatus>"
  BusOutput/226 -> Convert226/1  "<omega_WheelFR_radps>"
  debug_TET_s/1 -> Mux/269
  BusOutput/136 -> Convert136/1  "<res_dLoc1_m>"
  BusOutput/16 -> Convert16/1  "<Lat_FF_FIR_radpm>"
  Convert43/1 -> debug_mvdc_trajectory_driver_debug_Strategy_CommsStatus/1
  debug_VehicleSensorData_dTheta_PitchRateIMU1_radps/1 -> Mux/258
  Convert249/1 -> debug_VehicleSensorData_vy_CoGVel1_mps/1
  debug_mvdc_trajectory_driver_debug_EnablePathMatching/1 -> Mux/38
  Convert50/1 -> debug_mvdc_trajectory_driver_perf_ePeak_heading_rad/1
  BusOutput/40 -> Convert40/1  "<PathMatchingStatus>"
  BusOutput/39 -> Convert39/1  "<EnableDriving>"
  debug_mvdc_state_estimation_debug_Residuals_res_xLoc2_m/1 -> Mux/126
  debug_mvdc_trajectory_driver_debug_ParkBrakeActive/1 -> Mux/36
  debug_mvdc_state_estimation_debug_Diagnosis_fail_Loc1_b/1 -> Mux/145
  debug_mvdc_path_matching_debug_ActualPathPoint_DriveForce_N/1 -> Mux/35
  Convert31/1 -> debug_mvdc_path_matching_debug_ActualPathPoint_v_mps/1
  BusOutput/166 -> Convert166/1  "<EnableDriver>"
  BusOutput/36 -> Convert36/1  "<ParkBrakeActive>"
  BusOutput/138 -> Convert138/1  "<res_dLoc2_m>"
  debug_mvdc_trajectory_driver_debug_DriverStatus/1 -> Mux/37
  debug_mvdc_mue_estimation_delay_debug_Position_psi_rad/1 -> Mux/179
  BusOutput/268 -> Convert268/1  "<Time_s>"
  BusOutput/38 -> Convert38/1  "<EnablePathMatching>"
  debug_mvdc_path_matching_debug_ActualPathPoint_psi_rad/1 -> Mux/28
  debug_VehicleSensorData_valid_Wheelspeeds_b/1 -> Mux/229
  Convert262/1 -> debug_VehicleSensorData_ay_CoGIMU2_mps2/1
  Convert32/1 -> debug_mvdc_path_matching_debug_ActualPathPoint_ax_mps2/1
  BusOutput/33 -> Convert33/1  "<axFF_mps2>"
  debug_mvdc_path_matching_debug_ActualPathPoint_kappaFF_radpm/1 -> Mux/30
  BusOutput/32 -> Convert32/1  "<ax_mps2>"
  Convert204/1 -> debug_mvdc_mue_estimation_delay_debug_FX_MFtireforceRR_N/1
  debug_mvdc_mue_estimation_delay_debug_FY_MFtireforceFRmax_N/1 -> Mux/199
  BusOutput/30 -> Convert30/1  "<kappaFF_radpm>"
  BusOutput/11 -> Convert11/1  "<Lat_FB_Heading>"
  debug_mvdc_path_matching_debug_ActualPathPoint_x_m/1 -> Mux/26
  BusOutput/20 -> Convert20/1  "<s_m>"
  Convert20/1 -> debug_mvdc_path_matching_debug_PathPos_s_m/1
  BusOutput/22 -> Convert22/1  "<psi_rad>"
  debug_mvdc_mue_estimation_delay_debug_FY_MFtireforceFL_N/1 -> Mux/193
  debug_mvdc_path_matching_debug_PathPos_psi_rad/1 -> Mux/22
  BusOutput/220 -> Convert220/1  "<T_WheelRL_Nm>"
  Convert22/1 -> debug_mvdc_path_matching_debug_PathPos_psi_rad/1
  Convert139/1 -> debug_mvdc_state_estimation_debug_Diagnosis_valid_Loc1_b/1
  BusOutput/27 -> Convert27/1  "<y_m>"
  Convert25/1 -> debug_mvdc_path_matching_debug_ActualPathPoint_s_m/1
  Convert19/1 -> debug_mvdc_path_matching_debug_EmergencyTrajOK_b/1
  debug_VehicleSensorData_omega_WheelRL_radps/1 -> Mux/227
  Convert18/1 -> debug_mvdc_path_matching_debug_PerformanceTrajOK_b/1
  debug_VehicleSensorData_dPsi_YawRateIMU1_radps/1 -> Mux/259
  debug_mvdc_path_feedback_debug_Lat_LatPosError_m/1 -> Mux/12
  Convert13/1 -> debug_mvdc_path_feedback_debug_Lat_LatPosError_DerAna_mps/1
  Convert181/1 -> debug_mvdc_mue_estimation_delay_debug_FX_VehDynFR_N/1
  debug_mvdc_path_matching_debug_EmergencyTrajOK_b/1 -> Mux/19
  BusOutput/17 -> Convert17/1  "<Lat_all_KappaReq_radpm>"
  BusOutput/18 -> Convert18/1  "<PerformanceTrajOK_b>"
  BusOutput/265 -> Convert265/1  "<dTheta_PitchRateIMU2_radps>"
  BusOutput/169 -> Convert169/1  "<VehicleUnstable_b>"
  debug_mvdc_curvvel_tracking_debug_Req_Delta_rad/1 -> Mux/72
  BusOutput/12 -> Convert12/1  "<Lat_LatPosError_m>"
  BusOutput/14 -> Convert14/1  "<Lat_LatPosError_DerNum_mps>"
  debug_mvdc_path_feedback_debug_Lat_all_KappaReq_radpm/1 -> Mux/17
  Convert182/1 -> debug_mvdc_mue_estimation_delay_debug_FX_VehDynRL_N/1
  Convert108/1 -> debug_mvdc_state_estimation_debug_StateEstimate_psi_vel_rad/1
  BusOutput/159 -> Convert159/1  "<StateEstimation_Status>"
  Convert17/1 -> debug_mvdc_path_feedback_debug_Lat_all_KappaReq_radpm/1
  BusOutput/5 -> Convert5/1  "<BarriersR_y_m>"
  debug_mvdc_mue_estimation_delay_debug_FY_VehDynRR_N/1 -> Mux/187
  debug_mvdc_path_feedback_debug_Lat_LatPosError_DerAna_mps/1 -> Mux/13
  debug_mvdc_path_feedback_debug_BarriersL_y_m/1 -> Mux/3
  debug_mvdc_path_feedback_debug_BarriersR_x_m/1 -> Mux/4
  BusOutput/10 -> Convert10/1  "<Lat_FB_Position>"
  debug_mvdc_trajectory_driver_perf_LapTime_s/1 -> Mux/44
  BusOutput/177 -> Convert177/1  "<x_m>"
  debug_mvdc_path_feedback_debug_Lat_FB_Sum_KappaReq_radpm/1 -> Mux/9
  debugIn/1 -> BusOutput/1
  Convert9/1 -> debug_mvdc_path_feedback_debug_Lat_FB_Sum_KappaReq_radpm/1
  BusOutput/101 -> Convert101/1  "<dPsi_radps>"
  debug_mvdc_path_matching_debug_PathPos_s_m/1 -> Mux/20
  Convert149/1 -> debug_mvdc_state_estimation_debug_Diagnosis_fail_IMU1_b/1
  debug_VehicleSensorData_psi_YawAngleLoc1_rad/1 -> Mux/235
  BusOutput/49 -> Convert49/1  "<eRMS_heading_rad>"
  BusOutput/44 -> Convert44/1  "<LapTime_s>"
  BusOutput/21 -> Convert21/1  "<d_m>"
  Convert152/1 -> debug_mvdc_state_estimation_debug_Odom_Position_y_m/1
  debug_mvdc_curvvel_tracking_debug_Curv_FB_Diff_DeltaReq_rad/1 -> Mux/60
  debug_mvdc_state_estimation_debug_Odom_Position_y_m/1 -> Mux/152
  debug_mvdc_state_estimation_debug_Odom_Position_psi_rad/1 -> Mux/153
  debug_mvdc_state_estimation_debug_Diagnosis_valid_Loc1_b/1 -> Mux/139
  debug_mloc_diag_vehicle_debug_EstimatedCurrentPower_W/1 -> Mux/170
  Convert151/1 -> debug_mvdc_state_estimation_debug_Odom_Position_x_m/1
  debug_mvdc_state_estimation_debug_Diagnosis_fail_IMU1_b/1 -> Mux/149
  BusOutput/152 -> Convert152/1  "<y_m>"
  debug_mvdc_state_estimation_debug_Odom_Position_x_m/1 -> Mux/151
  Convert203/1 -> debug_mvdc_mue_estimation_delay_debug_FY_MFtireforceRLmax_N/1
  Convert197/1 -> debug_mvdc_mue_estimation_delay_debug_FY_MFtireforceFR_N/1
  Convert29/1 -> debug_mvdc_path_matching_debug_ActualPathPoint_kappa_radpm/1
  debug_mvdc_state_estimation_debug_Diagnosis_valid_Vel2_b/1 -> Mux/142
  debug_mvdc_path_feedback_debug_Lat_FB_Barriers/1 -> Mux/8
  debug_mvdc_state_estimation_debug_Diagnosis_valid_IMU2_b/1 -> Mux/144
  BusOutput/236 -> Convert236/1  "<t_EstimateLoc1_s>"
  BusOutput/119 -> Convert119/1  "<alphaFR_rad>"
  debug_ErrorCode/1 -> Mux/1
  debug_mvdc_trajectory_driver_debug_Strategy_Status/1 -> Mux/41
  BusOutput/258 -> Convert258/1  "<dTheta_PitchRateIMU1_radps>"
  debug_mvdc_state_estimation_debug_StateEstimate_ddPsi_radps2/1 -> Mux/111
  debug_mvdc_state_estimation_debug_StateEstimate_ax_mps2/1 -> Mux/106
  BusOutput/187 -> Convert187/1  "<FY_VehDynRR_N>"
  BusOutput/9 -> Convert9/1  "<Lat_FB_Sum_KappaReq_radpm>"
  Convert12/1 -> debug_mvdc_path_feedback_debug_Lat_LatPosError_m/1
  debug_mvdc_trajectory_driver_perf_e_lateral_m/1 -> Mux/45
  Convert143/1 -> debug_mvdc_state_estimation_debug_Diagnosis_valid_IMU1_b/1
  Convert28/1 -> debug_mvdc_path_matching_debug_ActualPathPoint_psi_rad/1
  Convert7/1 -> debug_mvdc_path_feedback_debug_RightDistance_m/1
  BusOutput/54 -> Convert54/1  "<e_kappa_radpm>"
  Convert144/1 -> debug_mvdc_state_estimation_debug_Diagnosis_valid_IMU2_b/1
  Convert172/1 -> debug_mvdc_mue_estimation_rt_debug_Position_x_m/1
  debug_mvdc_path_matching_debug_ActualPathPoint_kappa_radpm/1 -> Mux/29
  Convert101/1 -> debug_mvdc_state_estimation_debug_StateEstimate_dPsi_radps/1
  debug_VehicleSensorData_theta_PitchAngleLoc1_rad/1 -> Mux/234
  BusOutput/202 -> Convert202/1  "<FX_MFtireforceRLmax_N>"
  BusOutput/60 -> Convert60/1  "<Curv_FB_Diff_DeltaReq_rad>"
  BusOutput/62 -> Convert62/1  "<Curv_USComp_DeltaReq_rad>"
  Convert141/1 -> debug_mvdc_state_estimation_debug_Diagnosis_valid_Vel1_b/1
  BusOutput/110 -> Convert110/1  "<dBeta_radps>"
  BusOutput/162 -> Convert162/1  "<VehicleUnresponsive>"
  debug_mvdc_state_estimation_debug_Diagnosis_valid_Loc2_b/1 -> Mux/140
  Convert33/1 -> debug_mvdc_path_matching_debug_ActualPathPoint_axFF_mps2/1
  BusOutput/141 -> Convert141/1  "<valid_Vel1_b>"
  Convert118/1 -> debug_mvdc_state_estimation_debug_StateEstimate_alphaFL_rad/1
  Convert113/1 -> debug_mvdc_state_estimation_debug_StateEstimate_ay_vel_mps2/1
  Convert51/1 -> debug_mvdc_trajectory_driver_perf_e_v_mps/1
  debug_mvdc_state_estimation_debug_StateEstimate_vx_mps/1 -> Mux/102
  Convert140/1 -> debug_mvdc_state_estimation_debug_Diagnosis_valid_Loc2_b/1
  BusOutput/140 -> Convert140/1  "<valid_Loc2_b>"
  BusOutput/130 -> Convert130/1  "<res_vyVel1_mps>"
  debug_mvdc_curvvel_tracking_debug_Curv_USComp_DeltaReq_rad/1 -> Mux/62
  Convert55/1 -> debug_mvdc_trajectory_driver_perf_eRMS_kappa_radpm/1
  Convert95/1 -> debug_mvdc_state_estimation_debug_StateEstimate_Pos_x_m/1
  debug_mvdc_path_matching_debug_ActualPathPoint_v_mps/1 -> Mux/31
  debug_mvdc_state_estimation_debug_Residuals_res_yLoc1_m/1 -> Mux/124
  Convert86/1 -> debug_mvdc_exactlin_feedback_debug_LatAccTarget_mps2/1
  debug_mvdc_exactlin_feedback_debug_LatErrorDer_mps/1 -> Mux/85
  Convert137/1 -> debug_mvdc_state_estimation_debug_Residuals_res_sLoc2_m/1
  Convert66/1 -> debug_mvdc_curvvel_tracking_debug_Long_FF_Dist_FxReq_N/1
  BusOutput/134 -> Convert134/1  "<res_dPsi2_radps>"
  debug_mvdc_trajectory_driver_perf_ePeak_heading_rad/1 -> Mux/50
  debug_mvdc_state_estimation_debug_Residuals_res_dPsi1_radps/1 -> Mux/133
  Convert131/1 -> debug_mvdc_state_estimation_debug_Residuals_res_vxVel2_mps/1
  Convert135/1 -> debug_mvdc_state_estimation_debug_Residuals_res_sLoc1_m/1
  debug_mvdc_state_estimation_debug_Diagnosis_fail_IMU2_b/1 -> Mux/150
  BusOutput/131 -> Convert131/1  "<res_vxVel2_mps>"
  Convert119/1 -> debug_mvdc_state_estimation_debug_StateEstimate_alphaFR_rad/1
  BusOutput/24 -> Convert24/1  "<TrajCnt>"
  BusOutput/61 -> Convert61/1  "<Curv_FF_Kappa_DeltaReq_rad>"
  debug_mvdc_state_estimation_debug_Residuals_res_sLoc1_m/1 -> Mux/135
  debug_mvdc_path_feedback_debug_Lat_FB_Heading/1 -> Mux/11
  BusOutput/212 -> Convert212/1  "<TRFP_est_RLx>"
  BusOutput/25 -> Convert25/1  "<s_m>"
  BusOutput/241 -> Convert241/1  "<z_Loc2_m>"
  debug_mloc_statemachine_debug_VehicleReady2Drive/1 -> Mux/158
  BusOutput/167 -> Convert167/1  "<EnableHardEmergencyBrake>"
  Convert3/1 -> debug_mvdc_path_feedback_debug_BarriersL_y_m/1
  Convert115/1 -> debug_mvdc_state_estimation_debug_StateEstimate_lambdaFR_perc/1
  Convert127/1 -> debug_mvdc_state_estimation_debug_Residuals_res_yLoc2_m/1
  Convert205/1 -> debug_mvdc_mue_estimation_delay_debug_FY_MFtireforceRR_N/1
  Convert126/1 -> debug_mvdc_state_estimation_debug_Residuals_res_xLoc2_m/1
  BusOutput/126 -> Convert126/1  "<res_xLoc2_m>"
  Convert129/1 -> debug_mvdc_state_estimation_debug_Residuals_res_vxVel1_mps/1
  Convert102/1 -> debug_mvdc_state_estimation_debug_StateEstimate_vx_mps/1
  debug_mvdc_state_estimation_debug_StateEstimate_dPsi_radps/1 -> Mux/101
  debug_mvdc_path_feedback_debug_BarriersR_y_m/1 -> Mux/5
  Convert107/1 -> debug_mvdc_state_estimation_debug_StateEstimate_ay_mps2/1
  debug_mvdc_trajectory_driver_perf_ePeak_lateral_m/1 -> Mux/47
  Convert130/1 -> debug_mvdc_state_estimation_debug_Residuals_res_vyVel1_mps/1
  BusOutput/244 -> Convert244/1  "<psi_YawAngleLoc2_rad>"
  debug_mvdc_path_matching_debug_ActualPathPoint_LapCnt/1 -> Mux/23
  debug_mvdc_state_estimation_debug_Residuals_res_psiLoc2_rad/1 -> Mux/128
  debug_mvdc_exactlin_feedback_debug_LatError_m/1 -> Mux/84
  debug_mvdc_curvvel_tracking_debug_Curv_CurvError_radpm/1 -> Mux/63
  debug_mvdc_state_estimation_debug_Residuals_res_yLoc2_m/1 -> Mux/127
  BusOutput/223 -> Convert223/1  "<p_BrakeF_bar>"
  Convert111/1 -> debug_mvdc_state_estimation_debug_StateEstimate_ddPsi_radps2/1
  debug_mvdc_state_estimation_debug_Residuals_res_vyVel1_mps/1 -> Mux/130
  BusOutput/149 -> Convert149/1  "<fail_IMU1_b>"
  debug_mvdc_state_estimation_debug_Residuals_res_psiLoc1_rad/1 -> Mux/125
  debug_mvdc_state_estimation_debug_StateEstimate_alphaRR_rad/1 -> Mux/121
  Convert163/1 -> debug_mloc_statemachine_debug_TUMVehicleState/1
  Convert121/1 -> debug_mvdc_state_estimation_debug_StateEstimate_alphaRR_rad/1
  BusOutput/102 -> Convert102/1  "<vx_mps>"
  Convert116/1 -> debug_mvdc_state_estimation_debug_StateEstimate_lambdaRL_perc/1
  BusOutput/124 -> Convert124/1  "<res_yLoc1_m>"
  BusOutput/108 -> Convert108/1  "<psi_vel_rad>"
  BusOutput/41 -> Convert41/1  "<Strategy_Status>"
  Convert122/1 -> debug_mvdc_state_estimation_debug_StateEstimate_DiffFRAlpha_rad/1
  Convert106/1 -> debug_mvdc_state_estimation_debug_StateEstimate_ax_mps2/1
  BusOutput/129 -> Convert129/1  "<res_vxVel1_mps>"
  BusOutput/256 -> Convert256/1  "<az_CoGIMU1_mps2>"
  debug_mvdc_state_estimation_debug_StateEstimate_kappa_radpm/1 -> Mux/109
  Convert124/1 -> debug_mvdc_state_estimation_debug_Residuals_res_yLoc1_m/1
  BusOutput/122 -> Convert122/1  "<DiffFRAlpha_rad>"
  Convert26/1 -> debug_mvdc_path_matching_debug_ActualPathPoint_x_m/1
  BusOutput/55 -> Convert55/1  "<eRMS_kappa_radpm>"
  Convert175/1 -> debug_mvdc_mue_estimation_rt_debug_mue_estimation_AxleF/1
  debug_mvdc_state_estimation_debug_StateEstimate_alphaFR_rad/1 -> Mux/119
  Convert4/1 -> debug_mvdc_path_feedback_debug_BarriersR_x_m/1
  BusOutput/123 -> Convert123/1  "<res_xLoc1_m>"
  Convert112/1 -> debug_mvdc_state_estimation_debug_StateEstimate_ax_vel_mps2/1
  BusOutput/242 -> Convert242/1  "<phi_RollAngleLoc2_rad>"
  Convert208/1 -> debug_mvdc_mue_estimation_delay_debug_TRFP_est_FLx/1
  debug_mvdc_state_estimation_debug_StateEstimate_lambdaRR_perc/1 -> Mux/117
  debug_mvdc_mue_estimation_delay_debug_TRFP_est_RRy/1 -> Mux/215
  BusOutput/90 -> Convert90/1  "<EstimateFyR_N>"
  debug_mvdc_path_matching_debug_PerformanceTrajOK_b/1 -> Mux/18
  BusOutput/35 -> Convert35/1  "<DriveForce_N>"
  debug_VehicleSensorData_p_BrakeF_bar/1 -> Mux/223
  Convert220/1 -> debug_VehicleSensorData_T_WheelRL_Nm/1
  BusOutput/115 -> Convert115/1  "<lambdaFR_perc>"
  debug_VehicleSensorData_accuracy_Loc1/1 -> Mux/238
  debug_mvdc_state_estimation_debug_StateEstimate_dBeta_radps/1 -> Mux/110
  Convert268/1 -> debug_Time_s/1
  debug_mvdc_state_estimation_debug_StateEstimate_lambdaFL_perc/1 -> Mux/114
  BusOutput/8 -> Convert8/1  "<Lat_FB_Barriers>"
  BusOutput/114 -> Convert114/1  "<lambdaFL_perc>"
  BusOutput/135 -> Convert135/1  "<res_sLoc1_m>"
  BusOutput/1 -> Convert1/1  "<ErrorCode>"
  Convert248/1 -> debug_VehicleSensorData_vx_CoGVel1_mps/1
  BusOutput/113 -> Convert113/1  "<ay_vel_mps2>"
  BusOutput/112 -> Convert112/1  "<ax_vel_mps2>"
  debug_mvdc_state_estimation_debug_Residuals_res_xLoc1_m/1 -> Mux/123
  debug_VehicleSensorData_T_WheelRL_Nm/1 -> Mux/220
  BusOutput/120 -> Convert120/1  "<alphaRL_rad>"
  Convert2/1 -> debug_mvdc_path_feedback_debug_BarriersL_x_m/1
  Convert117/1 -> debug_mvdc_state_estimation_debug_StateEstimate_lambdaRR_perc/1
  BusOutput/34 -> Convert34/1  "<Delta_rad>"
  debug_mvdc_mue_estimation_delay_debug_FX_MFtireforceFRmax_N/1 -> Mux/198
  Convert232/1 -> debug_VehicleSensorData_z_Loc1_m/1
  debug_mvdc_state_estimation_debug_StateEstimate_alphaFL_rad/1 -> Mux/118
  Convert219/1 -> debug_VehicleSensorData_T_WheelFR_Nm/1
  BusOutput/106 -> Convert106/1  "<ax_mps2>"
  Convert38/1 -> debug_mvdc_trajectory_driver_debug_EnablePathMatching/1
  debug_mvdc_path_matching_debug_ActualPathPoint_TrajCnt/1 -> Mux/24
  BusOutput/176 -> Convert176/1  "<mue_estimation_AxleR>"
  Convert105/1 -> debug_mvdc_state_estimation_debug_StateEstimate_beta_rad/1
  Convert209/1 -> debug_mvdc_mue_estimation_delay_debug_TRFP_est_FLy/1
  Convert125/1 -> debug_mvdc_state_estimation_debug_Residuals_res_psiLoc1_rad/1
  BusOutput/103 -> Convert103/1  "<vy_mps>"
  debug_mvdc_path_feedback_debug_LeftDistance_m/1 -> Mux/6
  BusOutput/209 -> Convert209/1  "<TRFP_est_FLy>"
  Convert24/1 -> debug_mvdc_path_matching_debug_ActualPathPoint_TrajCnt/1
  debug_mvdc_curvvel_tracking_debug_Req_Fx_N/1 -> Mux/73
  debug_mvdc_path_matching_debug_ActualPathPoint_axFF_mps2/1 -> Mux/33
  Convert103/1 -> debug_mvdc_state_estimation_debug_StateEstimate_vy_mps/1
  debug_mvdc_trajectory_driver_perf_eRMS_lateral_m/1 -> Mux/46
  debug_mvdc_state_estimation_debug_StateEstimate_PosAccuracy/1 -> Mux/99
  Convert114/1 -> debug_mvdc_state_estimation_debug_StateEstimate_lambdaFL_perc/1
  debug_mvdc_state_estimation_debug_StateEstimate_v_mps/1 -> Mux/104
  Convert23/1 -> debug_mvdc_path_matching_debug_ActualPathPoint_LapCnt/1
  Convert30/1 -> debug_mvdc_path_matching_debug_ActualPathPoint_kappaFF_radpm/1
  BusOutput/13 -> Convert13/1  "<Lat_LatPosError_DerAna_mps>"
  debug_mvdc_state_estimation_debug_StateEstimate_psi_vel_rad/1 -> Mux/108
  Convert87/1 -> debug_mvdc_exactlin_feedback_debug_EstimateAlphaF_rad/1
  debug_mvdc_state_estimation_debug_Diagnosis_valid_IMU1_b/1 -> Mux/143
  Convert54/1 -> debug_mvdc_trajectory_driver_perf_e_kappa_radpm/1
  BusOutput/161 -> Convert161/1  "<Driver_Status>"
  BusOutput/250 -> Convert250/1  "<valid_Vel1_b>"
  BusOutput/261 -> Convert261/1  "<ax_CoGIMU2_mps2>"
  BusOutput/107 -> Convert107/1  "<ay_mps2>"
  Convert100/1 -> debug_mvdc_state_estimation_debug_StateEstimate_VelAccuracy/1
  debug_mvdc_state_estimation_debug_StateEstimate_ay_vel_mps2/1 -> Mux/113
  BusOutput/105 -> Convert105/1  "<beta_rad>"
  Convert97/1 -> debug_mvdc_state_estimation_debug_StateEstimate_Pos_psi_rad/1
  debug_VehicleSensorData_dPhi_RollRateIMU1_radps/1 -> Mux/257
  debug_mvdc_state_estimation_debug_StateEstimate_Pos_x_m/1 -> Mux/95
  BusOutput/26 -> Convert26/1  "<x_m>"
  debug_mvdc_trajectory_driver_debug_PathMatchingStatus/1 -> Mux/40
  BusOutput/95 -> Convert95/1  "<x_m>"
  Convert98/1 -> debug_mvdc_state_estimation_debug_StateEstimate_z_m/1
  debug_mvdc_state_estimation_debug_StateEstimate_SE_State/1 -> Mux/94
  debug_mvdc_mue_estimation_delay_debug_FX_VehDynRR_N/1 -> Mux/183
  BusOutput/2 -> Convert2/1  "<BarriersL_x_m>"
  BusOutput/15 -> Convert15/1  "<Lat_FF_Kappa_KappaReq_radpm>"
  debug_mvdc_path_feedback_debug_Lat_FB_Position/1 -> Mux/10
  debug_mvdc_state_estimation_debug_StateEstimate_z_m/1 -> Mux/98
  Convert120/1 -> debug_mvdc_state_estimation_debug_StateEstimate_alphaRL_rad/1
  BusOutput/253 -> Convert253/1  "<valid_Vel2_b>"
  Convert99/1 -> debug_mvdc_state_estimation_debug_StateEstimate_PosAccuracy/1
  Convert212/1 -> debug_mvdc_mue_estimation_delay_debug_TRFP_est_RLx/1
  debug_mvdc_state_estimation_debug_Diagnosis_fail_Vel2_b/1 -> Mux/148
  BusOutput/116 -> Convert116/1  "<lambdaRL_perc>"
  Convert8/1 -> debug_mvdc_path_feedback_debug_Lat_FB_Barriers/1
  debug_mvdc_state_estimation_debug_StateEstimate_Pos_y_m/1 -> Mux/96
  BusOutput/137 -> Convert137/1  "<res_sLoc2_m>"
  BusOutput/99 -> Convert99/1  "<PosAccuracy>"
  BusOutput/121 -> Convert121/1  "<alphaRR_rad>"
  debug_mvdc_mue_estimation_delay_debug_TRFP_est_FRx/1 -> Mux/210
  debug_mvdc_path_matching_debug_ActualPathPoint_s_m/1 -> Mux/25
  Convert83/1 -> debug_mvdc_exactlin_feedback_debug_LongAccTarget_mps2/1
  debug_mvdc_state_estimation_debug_StateEstimate_Pos_psi_rad/1 -> Mux/97
  Convert215/1 -> debug_mvdc_mue_estimation_delay_debug_TRFP_est_RRy/1
  debug_mvdc_exactlin_feedback_debug_RequestDelta_rad/1 -> Mux/91
  debug_VehicleSensorData_z_Loc1_m/1 -> Mux/232
  Convert241/1 -> debug_VehicleSensorData_z_Loc2_m/1
  debug_mvdc_trajectory_driver_perf_ePeak_v_mps/1 -> Mux/53
  BusOutput/94 -> Convert94/1  "<SE_State>"
  BusOutput/23 -> Convert23/1  "<LapCnt>"
  debug_mvdc_exactlin_feedback_debug_EstimateFyR_N/1 -> Mux/90
  Convert94/1 -> debug_mvdc_state_estimation_debug_StateEstimate_SE_State/1
  Convert92/1 -> debug_mvdc_exactlin_feedback_debug_RequestFx_N/1
  debug_mvdc_mue_estimation_delay_debug_FX_MFtireforceFLmax_N/1 -> Mux/194
  Convert90/1 -> debug_mvdc_exactlin_feedback_debug_EstimateFyR_N/1
  BusOutput/31 -> Convert31/1  "<v_mps>"
  Convert91/1 -> debug_mvdc_exactlin_feedback_debug_RequestDelta_rad/1
  debug_mvdc_state_estimation_debug_StateEstimate_SE_Status/1 -> Mux/93
  debug_mvdc_mue_estimation_delay_debug_FZ_VehDynFR_N/1 -> Mux/189
  Convert53/1 -> debug_mvdc_trajectory_driver_perf_ePeak_v_mps/1
  BusOutput/84 -> Convert84/1  "<LatError_m>"
  debug_mvdc_exactlin_feedback_debug_EstimateAlphaR_rad/1 -> Mux/88
  BusOutput/91 -> Convert91/1  "<RequestDelta_rad>"
  debug_mvdc_exactlin_feedback_debug_EstimateFyF_N/1 -> Mux/89
  Convert93/1 -> debug_mvdc_state_estimation_debug_StateEstimate_SE_Status/1
  Convert257/1 -> debug_VehicleSensorData_dPhi_RollRateIMU1_radps/1
  Convert41/1 -> debug_mvdc_trajectory_driver_debug_Strategy_Status/1
  BusOutput/6 -> Convert6/1  "<LeftDistance_m>"
  BusOutput/96 -> Convert96/1  "<y_m>"
  debug_mvdc_mue_estimation_delay_debug_FZ_VehDynRL_N/1 -> Mux/190
  debug_mvdc_trajectory_driver_perf_eRMS_heading_rad/1 -> Mux/49
  debug_mvdc_exactlin_feedback_debug_LatAccTarget_mps2/1 -> Mux/86
  debug_mvdc_curvvel_tracking_debug_EnableEmergency/1 -> Mux/76
  debug_mvdc_exactlin_feedback_debug_LongAccTarget_mps2/1 -> Mux/83
  BusOutput/231 -> Convert231/1  "<y_Loc1_m>"
  Convert142/1 -> debug_mvdc_state_estimation_debug_Diagnosis_valid_Vel2_b/1
  Convert21/1 -> debug_mvdc_path_matching_debug_PathPos_d_m/1
  debug_mloc_statemachine_debug_StateEstimation_Status/1 -> Mux/159
  Convert138/1 -> debug_mvdc_state_estimation_debug_Residuals_res_dLoc2_m/1
  debug_mvdc_state_estimation_debug_Residuals_res_sLoc2_m/1 -> Mux/137
  Convert85/1 -> debug_mvdc_exactlin_feedback_debug_LatErrorDer_mps/1
  debug_mvdc_curvvel_tracking_debug_Curv_TargetAy_mps2/1 -> Mux/57
  BusOutput/190 -> Convert190/1  "<FZ_VehDynRL_N>"
  BusOutput/47 -> Convert47/1  "<ePeak_lateral_m>"
  debug_mvdc_mue_estimation_delay_debug_FX_MFtireforceFL_N/1 -> Mux/192
  BusOutput/87 -> Convert87/1  "<EstimateAlphaF_rad>"
  Convert254/1 -> debug_VehicleSensorData_ax_CoGIMU1_mps2/1
  BusOutput/83 -> Convert83/1  "<LongAccTarget_mps2>"
  debug_VehicleSensorData_valid_Vel1_b/1 -> Mux/250
  BusOutput/37 -> Convert37/1  "<DriverStatus>"
  Convert236/1 -> debug_VehicleSensorData_t_EstimateLoc1_s/1
  debug_mvdc_exactlin_feedback_debug_EstimateAlphaF_rad/1 -> Mux/87
  debug_mvdc_state_estimation_debug_StateEstimate_beta_rad/1 -> Mux/105
  Convert14/1 -> debug_mvdc_path_feedback_debug_Lat_LatPosError_DerNum_mps/1
  Convert79/1 -> debug_mvdc_curvvel_tracking_debug_TCProportionalForce_N/1
  BusOutput/173 -> Convert173/1  "<y_m>"
  Convert65/1 -> debug_mvdc_curvvel_tracking_debug_Long_FB_Dist_FxReq_N/1
  Convert193/1 -> debug_mvdc_mue_estimation_delay_debug_FY_MFtireforceFL_N/1
  debug_mvdc_state_estimation_debug_StateEstimate_lambdaRL_perc/1 -> Mux/116
  BusOutput/78 -> Convert78/1  "<TCSlipDifference_perc>"
  BusOutput/260 -> Convert260/1  "<valid_IMU1_b>"
  Convert81/1 -> debug_mvdc_curvvel_tracking_debug_MaximumLongForce_N/1
  Convert34/1 -> debug_mvdc_path_matching_debug_ActualPathPoint_Delta_rad/1
  BusOutput/89 -> Convert89/1  "<EstimateFyF_N>"
  Convert146/1 -> debug_mvdc_state_estimation_debug_Diagnosis_fail_Loc2_b/1
  debug_mloc_statemachine_debug_TUMVehicleState/1 -> Mux/163
  debug_mvdc_state_estimation_debug_Residuals_res_dPsi2_radps/1 -> Mux/134
  debug_mvdc_curvvel_tracking_debug_TCSlipDifference_perc/1 -> Mux/78
  BusOutput/45 -> Convert45/1  "<e_lateral_m>"
  Convert82/1 -> debug_mvdc_exactlin_feedback_debug_VelocityError_mps/1
  debug_mvdc_curvvel_tracking_debug_MaximumLongForce_N/1 -> Mux/81
  BusOutput/29 -> Convert29/1  "<kappa_radpm>"
  BusOutput/93 -> Convert93/1  "<SE_Status>"
  debug_mvdc_path_feedback_debug_RightDistance_m/1 -> Mux/7
  debug_mvdc_curvvel_tracking_debug_TCCorrectiveForce_N/1 -> Mux/77
  BusOutput/85 -> Convert85/1  "<LatErrorDer_mps>"
  debug_mvdc_state_estimation_debug_Residuals_res_vxVel1_mps/1 -> Mux/129
  Convert1/1 -> debug_ErrorCode/1
  debug_mvdc_mue_estimation_rt_debug_mue_estimation_AxleF/1 -> Mux/175
  debug_mvdc_mue_estimation_delay_debug_FX_MFtireforceFR_N/1 -> Mux/196
  Convert165/1 -> debug_mloc_statemachine_debug_EnableControlOutputs/1
  debug_mvdc_curvvel_tracking_debug_ControlState/1 -> Mux/74
  debug_mvdc_curvvel_tracking_debug_Long_axTarget_mps2/1 -> Mux/71
  debug_VehicleSensorData_valid_IMU2_b/1 -> Mux/267
  Convert75/1 -> debug_mvdc_curvvel_tracking_debug_EnableDriving/1
  Convert78/1 -> debug_mvdc_curvvel_tracking_debug_TCSlipDifference_perc/1
  debug_mvdc_mue_estimation_delay_debug_TRFP_est_RRx/1 -> Mux/214
  BusOutput/175 -> Convert175/1  "<mue_estimation_AxleF>"
  Convert183/1 -> debug_mvdc_mue_estimation_delay_debug_FX_VehDynRR_N/1
  Convert76/1 -> debug_mvdc_curvvel_tracking_debug_EnableEmergency/1
  BusOutput/73 -> Convert73/1  "<Req_Fx_N>"
  BusOutput/77 -> Convert77/1  "<TCCorrectiveForce_N>"
  Convert237/1 -> debug_VehicleSensorData_valid_Loc1_b/1
  debug_VehicleSensorData_ay_CoGIMU1_mps2/1 -> Mux/255
  BusOutput/88 -> Convert88/1  "<EstimateAlphaR_rad>"
  BusOutput/4 -> Convert4/1  "<BarriersR_x_m>"
  debug_mvdc_curvvel_tracking_debug_EnableDriving/1 -> Mux/75
  Convert89/1 -> debug_mvdc_exactlin_feedback_debug_EstimateFyF_N/1
  debug_mvdc_mue_estimation_delay_debug_TRFP_est_FLy/1 -> Mux/209
  Convert64/1 -> debug_mvdc_curvvel_tracking_debug_Curv_TargetCurv_radpm/1
  debug_mvdc_path_matching_debug_ActualPathPoint_y_m/1 -> Mux/27
  Convert174/1 -> debug_mvdc_mue_estimation_rt_debug_Position_psi_rad/1
  Convert72/1 -> debug_mvdc_curvvel_tracking_debug_Req_Delta_rad/1
  BusOutput/74 -> Convert74/1  "<ControlState>"
  BusOutput/72 -> Convert72/1  "<Req_Delta_rad>"
  debug_VehicleSensorData_vx_CoGVel2_mps/1 -> Mux/251
  BusOutput/196 -> Convert196/1  "<FX_MFtireforceFR_N>"
  Convert71/1 -> debug_mvdc_curvvel_tracking_debug_Long_axTarget_mps2/1
  debug_mvdc_mue_estimation_delay_debug_FY_MFtireforceRL_N/1 -> Mux/201
  debug_mvdc_exactlin_feedback_debug_VelocityError_mps/1 -> Mux/82
  BusOutput/70 -> Convert70/1  "<Long_TargetSpeed_mps>"
  BusOutput/204 -> Convert204/1  "<FX_MFtireforceRR_N>"
  debug_mvdc_path_feedback_debug_Lat_FF_FIR_radpm/1 -> Mux/16
  Convert68/1 -> debug_mvdc_curvvel_tracking_debug_Long_FF_Traj_FxReq_N/1
  Convert136/1 -> debug_mvdc_state_estimation_debug_Residuals_res_dLoc1_m/1
  BusOutput/75 -> Convert75/1  "<EnableDriving>"
  BusOutput/82 -> Convert82/1  "<VelocityError_mps>"
  BusOutput/53 -> Convert53/1  "<ePeak_v_mps>"
  debug_mvdc_curvvel_tracking_debug_Long_FB_Dist_FxReq_N/1 -> Mux/65
  Convert84/1 -> debug_mvdc_exactlin_feedback_debug_LatError_m/1
  Convert145/1 -> debug_mvdc_state_estimation_debug_Diagnosis_fail_Loc1_b/1
  Convert179/1 -> debug_mvdc_mue_estimation_delay_debug_Position_psi_rad/1
  debug_mvdc_curvvel_tracking_debug_Long_FF_Dist_FxReq_N/1 -> Mux/66
  debug_mloc_statemachine_debug_Driver_Status/1 -> Mux/161
  Convert27/1 -> debug_mvdc_path_matching_debug_ActualPathPoint_y_m/1
  Convert210/1 -> debug_mvdc_mue_estimation_delay_debug_TRFP_est_FRx/1
  BusOutput/67 -> Convert67/1  "<Long_FB_VelDiff_FxReq_N>"
  debug_mvdc_state_estimation_debug_Residuals_res_dLoc2_m/1 -> Mux/138
  debug_mvdc_curvvel_tracking_debug_Long_VelError_mps/1 -> Mux/69
  Convert56/1 -> debug_mvdc_trajectory_driver_perf_ePeak_kappa_radpm/1
  debug_mvdc_curvvel_tracking_debug_Long_FB_VelDiff_FxReq_N/1 -> Mux/67
  BusOutput/79 -> Convert79/1  "<TCProportionalForce_N>"
  Convert5/1 -> debug_mvdc_path_feedback_debug_BarriersR_y_m/1
  BusOutput/71 -> Convert71/1  "<Long_axTarget_mps2>"
  BusOutput/64 -> Convert64/1  "<Curv_TargetCurv_radpm>"
  Convert69/1 -> debug_mvdc_curvvel_tracking_debug_Long_VelError_mps/1
  debug_mvdc_curvvel_tracking_debug_TCProportionalForce_N/1 -> Mux/79
  Convert11/1 -> debug_mvdc_path_feedback_debug_Lat_FB_Heading/1
  BusOutput/66 -> Convert66/1  "<Long_FF_Dist_FxReq_N>"
  BusOutput/69 -> Convert69/1  "<Long_VelError_mps>"
  debug_mvdc_curvvel_tracking_debug_Long_FF_Traj_FxReq_N/1 -> Mux/68
  BusOutput/237 -> Convert237/1  "<valid_Loc1_b>"
  Convert88/1 -> debug_mvdc_exactlin_feedback_debug_EstimateAlphaR_rad/1
  debug_VehicleSensorData_T_WheelRR_Nm/1 -> Mux/221
  debug_mvdc_path_matching_debug_ActualPathPoint_Delta_rad/1 -> Mux/34
  BusOutput/188 -> Convert188/1  "<FZ_VehDynFL_N>"
  Convert67/1 -> debug_mvdc_curvvel_tracking_debug_Long_FB_VelDiff_FxReq_N/1
  debug_VehicleSensorData_phi_RollAngleLoc2_rad/1 -> Mux/242
  debug_mvdc_curvvel_tracking_debug_Long_TargetSpeed_mps/1 -> Mux/70
  BusOutput/56 -> Convert56/1  "<ePeak_kappa_radpm>"
  debug_mvdc_mue_estimation_rt_debug_Position_x_m/1 -> Mux/172
  BusOutput/48 -> Convert48/1  "<e_heading_rad>"
  Convert169/1 -> debug_mloc_diag_vehicle_debug_VehicleUnstable_b/1
  debug_VehicleSensorData_x_Loc2_m/1 -> Mux/239
  Convert207/1 -> debug_mvdc_mue_estimation_delay_debug_FY_MFtireforceRRmax_N/1
  BusOutput/68 -> Convert68/1  "<Long_FF_Traj_FxReq_N>"
